simulink model "model_compatible"  (Simulink 7.5)
(part 1 of 2)
settings: Solver=ode45  StartTime=0.0  StopTime=10.0  RelTol=1e-3
libraries: powerlib x223
settings Model: Creator=lej  LastModifiedBy=epezhman  CovModelRefEnable=off
settings DataIOCC: SaveFormat=StructureWithTime
settings OptimizationCC: ExpressionDepthLimit=128
settings DebuggingCC: UnderspecifiedInitializationDetection=Simplified  MergeDetectMultiDrivingBlocksExec=error  SolverPrmCheckMsg=none  FcnCallInpInsideContextMsg=Enable All  StateNameClashWarn=none
settings HardwareCC: ProdIntDivRoundTo=Zero  ProdEndianess=LittleEndian  ProdHWDeviceType=Specified
settings CodeAppCC: CustomSymbolStrType=$N$R$M_T
settings GRTTargetCC: TargetFunctionLibrary=C89/C90 (ANSI)  GeneratePreprocessorConditionals=Use local settings

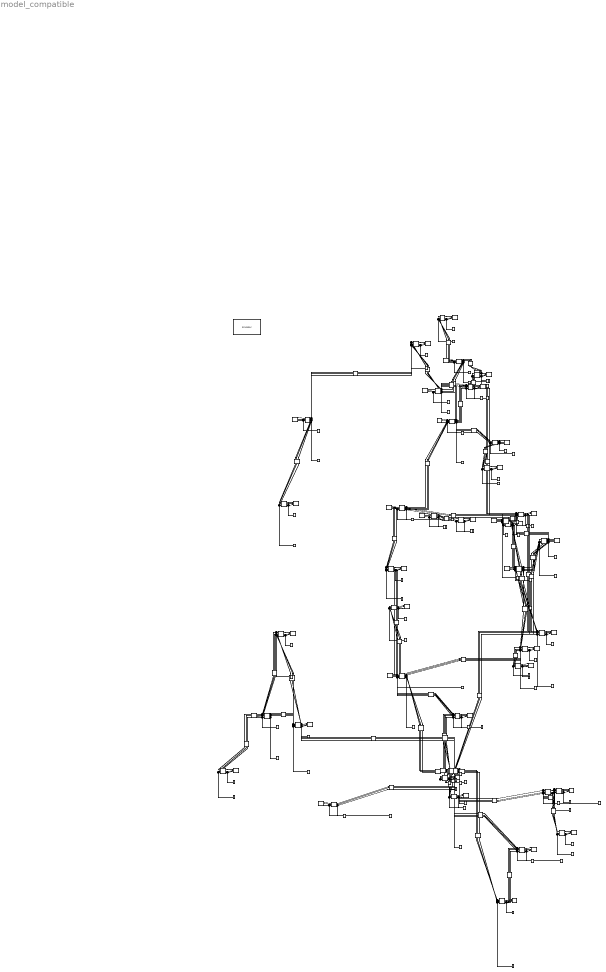
== system model_compatible ==
  note: 150000 Volts Power Line
  note: 225000 Volts Power Line
  DIV_225_Kv_MORNAGUIA_(_MNIHLA_1_BIR_MCHARGA)_CN_129996167_225000_CN_125504235_225000 : powerlib/Elements/Distributed Parameters Line  Phases=3  Frequency=50  Resistance=[0.01273 0.3864]  Inductance="[0.9337e-3  4.1264e-3]"  Capacitance=[12.74e-9 7.751e-9]  Length=112.5736  x1=[8.73114913702011e-11 380000 380000;314.159265358979 314.159265358979 314.159265358979;-0.177670123217348 0.415246442777429 -1.15554988401747]  x2=[1.26090477118469e-09 381852.398472139 381852.398472139;314.159265358979 314.159265358979 314.159265358979;-1.41941675517191 0.415007521738739 -1.15578880505616]  x3=[1.07663708898761e-11 1405.24743813465 1405.24743813466;314.159265358979 314.159265358979 314.159265358979;-2.70558821102223 0.316110507002444 -1.25468581979246]  x4=[8.62234243168895e-12 1405.96374414071 1405.9637441407;314.159265358979 314.159265358979 314.159265358979;0.245769282942371 0.405640215255436 -1.16515611153945]  x5=0.000565541566995742  V1=ones(3,3)  V2=ones(3,3)  I1=ones(3,3)  I2=ones(3,3)  nHarmo=1  Measurements=None
  G_93164455_ : powerlib/Electrical Sources/Three-Phase Source  InternalConnection=Yg  VoltagePhases=off  Voltage=225000  PhaseAngle=0  Voltage_phases=[ 1 1 1]*380000  PhaseAngles_phases=[ 0 0 0]  Frequency=50  NonIdealSource=on  SpecifyImpedance=off  Resistance=0.8929  Inductance=16.58e-3  ShortCircuitLevel=100e6  BaseVoltage=225000  XRratio=7  BusType=swing  Pref=10e3  Qref=0  Prefabc=[3333.33 3333.33 3333.33]  Qrefabc=[0 0 0]  Qmin=-inf  Qmax=inf
  LIGNE_150_KV_METLAOUI_DIV_MDHILLA_CN_206389818_150000_CN_206449367_150000 : powerlib/Elements/Distributed Parameters Line  Phases=3  Frequency=50  Resistance=[0.01273 0.3864]  Inductance="[0.9337e-3  4.1264e-3]"  Capacitance=[12.74e-9 7.751e-9]  Length=32.7201  x1=[8.73114913702011e-11 380000 380000;314.159265358979 314.159265358979 314.159265358979;-0.177670123217348 0.415246442777429 -1.15554988401747]  x2=[1.26090477118469e-09 381852.398472139 381852.398472139;314.159265358979 314.159265358979 314.159265358979;-1.41941675517191 0.415007521738739 -1.15578880505616]  x3=[1.07663708898761e-11 1405.24743813465 1405.24743813466;314.159265358979 314.159265358979 314.159265358979;-2.70558821102223 0.316110507002444 -1.25468581979246]  x4=[8.62234243168895e-12 1405.96374414071 1405.9637441407;314.159265358979 314.159265358979 314.159265358979;0.245769282942371 0.405640215255436 -1.16515611153945]  x5=0.000565541566995742  V1=ones(3,3)  V2=ones(3,3)  I1=ones(3,3)  I2=ones(3,3)  nHarmo=1  Measurements=None
  LIGNE_150_KV_METLAOUI_TOZEUR_CN_207339172_150000_CN_206389818_150000 : powerlib/Elements/Distributed Parameters Line  Phases=3  Frequency=50  Resistance=[0.01273 0.3864]  Inductance="[0.9337e-3  4.1264e-3]"  Capacitance=[12.74e-9 7.751e-9]  Length=61.5655  x1=[8.73114913702011e-11 380000 380000;314.159265358979 314.159265358979 314.159265358979;-0.177670123217348 0.415246442777429 -1.15554988401747]  x2=[1.26090477118469e-09 381852.398472139 381852.398472139;314.159265358979 314.159265358979 314.159265358979;-1.41941675517191 0.415007521738739 -1.15578880505616]  x3=[1.07663708898761e-11 1405.24743813465 1405.24743813466;314.159265358979 314.159265358979 314.159265358979;-2.70558821102223 0.316110507002444 -1.25468581979246]  x4=[8.62234243168895e-12 1405.96374414071 1405.9637441407;314.159265358979 314.159265358979 314.159265358979;0.245769282942371 0.405640215255436 -1.16515611153945]  x5=0.000565541566995742  V1=ones(3,3)  V2=ones(3,3)  I1=ones(3,3)  I2=ones(3,3)  nHarmo=1  Measurements=None
  LIGNE_150_Kv_BOUCHEMMA_CIMENTERIE_DE_GABES_CN_322419513_150000_CN_189193656_150000 : powerlib/Elements/Distributed Parameters Line  Phases=3  Frequency=50  Resistance=[0.01273 0.3864]  Inductance="[0.9337e-3  4.1264e-3]"  Capacitance=[12.74e-9 7.751e-9]  Length=6.701  x1=[8.73114913702011e-11 380000 380000;314.159265358979 314.159265358979 314.159265358979;-0.177670123217348 0.415246442777429 -1.15554988401747]  x2=[1.26090477118469e-09 381852.398472139 381852.398472139;314.159265358979 314.159265358979 314.159265358979;-1.41941675517191 0.415007521738739 -1.15578880505616]  x3=[1.07663708898761e-11 1405.24743813465 1405.24743813466;314.159265358979 314.159265358979 314.159265358979;-2.70558821102223 0.316110507002444 -1.25468581979246]  x4=[8.62234243168895e-12 1405.96374414071 1405.9637441407;314.159265358979 314.159265358979 314.159265358979;0.245769282942371 0.405640215255436 -1.16515611153945]  x5=0.000565541566995742  V1=ones(3,3)  V2=ones(3,3)  I1=ones(3,3)  I2=ones(3,3)  nHarmo=1  Measurements=None
  LIGNE_150_Kv_BOUCHEMMA_GABES_SUD_CN_189193656_150000_CN_242392536_150000 : powerlib/Elements/Distributed Parameters Line  Phases=3  Frequency=50  Resistance=[0.01273 0.3864]  Inductance="[0.9337e-3  4.1264e-3]"  Capacitance=[12.74e-9 7.751e-9]  Length=21.5599  x1=[8.73114913702011e-11 380000 380000;314.159265358979 314.159265358979 314.159265358979;-0.177670123217348 0.415246442777429 -1.15554988401747]  x2=[1.26090477118469e-09 381852.398472139 381852.398472139;314.159265358979 314.159265358979 314.159265358979;-1.41941675517191 0.415007521738739 -1.15578880505616]  x3=[1.07663708898761e-11 1405.24743813465 1405.24743813466;314.159265358979 314.159265358979 314.159265358979;-2.70558821102223 0.316110507002444 -1.25468581979246]  x4=[8.62234243168895e-12 1405.96374414071 1405.9637441407;314.159265358979 314.159265358979 314.159265358979;0.245769282942371 0.405640215255436 -1.16515611153945]  x5=0.000565541566995742  V1=ones(3,3)  V2=ones(3,3)  I1=ones(3,3)  I2=ones(3,3)  nHarmo=1  Measurements=None
  LIGNE_150_Kv_BOUCHEMMA_KEBILI_CN_189193656_150000_CN_253586233_150000 : powerlib/Elements/Distributed Parameters Line  Phases=3  Frequency=50  Resistance=[0.01273 0.3864]  Inductance="[0.9337e-3  4.1264e-3]"  Capacitance=[12.74e-9 7.751e-9]  Length=83.1245  x1=[8.73114913702011e-11 380000 380000;314.159265358979 314.159265358979 314.159265358979;-0.177670123217348 0.415246442777429 -1.15554988401747]  x2=[1.26090477118469e-09 381852.398472139 381852.398472139;314.159265358979 314.159265358979 314.159265358979;-1.41941675517191 0.415007521738739 -1.15578880505616]  x3=[1.07663708898761e-11 1405.24743813465 1405.24743813466;314.159265358979 314.159265358979 314.159265358979;-2.70558821102223 0.316110507002444 -1.25468581979246]  x4=[8.62234243168895e-12 1405.96374414071 1405.9637441407;314.159265358979 314.159265358979 314.159265358979;0.245769282942371 0.405640215255436 -1.16515611153945]  x5=0.000565541566995742  V1=ones(3,3)  V2=ones(3,3)  I1=ones(3,3)  I2=ones(3,3)  nHarmo=1  Measurements=None
  LIGNE_150_Kv_DIV_SKHIRA_CN_202286224_150000_CN_189193656_150000 : powerlib/Elements/Distributed Parameters Line  Phases=3  Frequency=50  Resistance=[0.01273 0.3864]  Inductance="[0.9337e-3  4.1264e-3]"  Capacitance=[12.74e-9 7.751e-9]  Length=63.8559  x1=[8.73114913702011e-11 380000 380000;314.159265358979 314.159265358979 314.159265358979;-0.177670123217348 0.415246442777429 -1.15554988401747]  x2=[1.26090477118469e-09 381852.398472139 381852.398472139;314.159265358979 314.159265358979 314.159265358979;-1.41941675517191 0.415007521738739 -1.15578880505616]  x3=[1.07663708898761e-11 1405.24743813465 1405.24743813466;314.159265358979 314.159265358979 314.159265358979;-2.70558821102223 0.316110507002444 -1.25468581979246]  x4=[8.62234243168895e-12 1405.96374414071 1405.9637441407;314.159265358979 314.159265358979 314.159265358979;0.245769282942371 0.405640215255436 -1.16515611153945]  x5=0.000565541566995742  V1=ones(3,3)  V2=ones(3,3)  I1=ones(3,3)  I2=ones(3,3)  nHarmo=1  Measurements=None
  LIGNE_150_Kv_DIV_SKHIRA_CN_202286224_150000_CN_201812735_150000 : powerlib/Elements/Distributed Parameters Line  Phases=3  Frequency=50  Resistance=[0.01273 0.3864]  Inductance="[0.9337e-3  4.1264e-3]"  Capacitance=[12.74e-9 7.751e-9]  Length=60.8483  x1=[8.73114913702011e-11 380000 380000;314.159265358979 314.159265358979 314.159265358979;-0.177670123217348 0.415246442777429 -1.15554988401747]  x2=[1.26090477118469e-09 381852.398472139 381852.398472139;314.159265358979 314.159265358979 314.159265358979;-1.41941675517191 0.415007521738739 -1.15578880505616]  x3=[1.07663708898761e-11 1405.24743813465 1405.24743813466;314.159265358979 314.159265358979 314.159265358979;-2.70558821102223 0.316110507002444 -1.25468581979246]  x4=[8.62234243168895e-12 1405.96374414071 1405.9637441407;314.159265358979 314.159265358979 314.159265358979;0.245769282942371 0.405640215255436 -1.16515611153945]  x5=0.000565541566995742  V1=ones(3,3)  V2=ones(3,3)  I1=ones(3,3)  I2=ones(3,3)  nHarmo=1  Measurements=None
  LIGNE_150_Kv_DIV_SKHIRA_CN_202286224_150000_CN_242390602_150000 : powerlib/Elements/Distributed Parameters Line  Phases=3  Frequency=50  Resistance=[0.01273 0.3864]  Inductance="[0.9337e-3  4.1264e-3]"  Capacitance=[12.74e-9 7.751e-9]  Length=66.6914  x1=[8.73114913702011e-11 380000 380000;314.159265358979 314.159265358979 314.159265358979;-0.177670123217348 0.415246442777429 -1.15554988401747]  x2=[1.26090477118469e-09 381852.398472139 381852.398472139;314.159265358979 314.159265358979 314.159265358979;-1.41941675517191 0.415007521738739 -1.15578880505616]  x3=[1.07663708898761e-11 1405.24743813465 1405.24743813466;314.159265358979 314.159265358979 314.159265358979;-2.70558821102223 0.316110507002444 -1.25468581979246]  x4=[8.62234243168895e-12 1405.96374414071 1405.9637441407;314.159265358979 314.159265358979 314.159265358979;0.245769282942371 0.405640215255436 -1.16515611153945]  x5=0.000565541566995742  V1=ones(3,3)  V2=ones(3,3)  I1=ones(3,3)  I2=ones(3,3)  nHarmo=1  Measurements=None
  LIGNE_150_Kv_ENFIDHA_DIV_BOUFICHA_CN_131220525_150000_CN_106469430_150000 : powerlib/Elements/Distributed Parameters Line  Phases=3  Frequency=50  Resistance=[0.01273 0.3864]  Inductance="[0.9337e-3  4.1264e-3]"  Capacitance=[12.74e-9 7.751e-9]  Length=29.2926  x1=[8.73114913702011e-11 380000 380000;314.159265358979 314.159265358979 314.159265358979;-0.177670123217348 0.415246442777429 -1.15554988401747]  x2=[1.26090477118469e-09 381852.398472139 381852.398472139;314.159265358979 314.159265358979 314.159265358979;-1.41941675517191 0.415007521738739 -1.15578880505616]  x3=[1.07663708898761e-11 1405.24743813465 1405.24743813466;314.159265358979 314.159265358979 314.159265358979;-2.70558821102223 0.316110507002444 -1.25468581979246]  x4=[8.62234243168895e-12 1405.96374414071 1405.9637441407;314.159265358979 314.159265358979 314.159265358979;0.245769282942371 0.405640215255436 -1.16515611153945]  x5=0.000565541566995742  V1=ones(3,3)  V2=ones(3,3)  I1=ones(3,3)  I2=ones(3,3)  nHarmo=1  Measurements=None
  LIGNE_150_Kv_MEKNASSY_HAJEB_LAYOUN_CN_224417135_225000_CN_201812735_225000 : powerlib/Elements/Distributed Parameters Line  Phases=3  Frequency=50  Resistance=[0.01273 0.3864]  Inductance="[0.9337e-3  4.1264e-3]"  Capacitance=[12.74e-9 7.751e-9]  Length=81.6177  x1=[8.73114913702011e-11 380000 380000;314.159265358979 314.159265358979 314.159265358979;-0.177670123217348 0.415246442777429 -1.15554988401747]  x2=[1.26090477118469e-09 381852.398472139 381852.398472139;314.159265358979 314.159265358979 314.159265358979;-1.41941675517191 0.415007521738739 -1.15578880505616]  x3=[1.07663708898761e-11 1405.24743813465 1405.24743813466;314.159265358979 314.159265358979 314.159265358979;-2.70558821102223 0.316110507002444 -1.25468581979246]  x4=[8.62234243168895e-12 1405.96374414071 1405.9637441407;314.159265358979 314.159265358979 314.159265358979;0.245769282942371 0.405640215255436 -1.16515611153945]  x5=0.000565541566995742  V1=ones(3,3)  V2=ones(3,3)  I1=ones(3,3)  I2=ones(3,3)  nHarmo=1  Measurements=None
  LIGNE_150_Kv_MEKNASSY_SIDI_BOUZID_CN_174150822_150000_CN_201812735_150000 : powerlib/Elements/Distributed Parameters Line  Phases=3  Frequency=50  Resistance=[0.01273 0.3864]  Inductance="[0.9337e-3  4.1264e-3]"  Capacitance=[12.74e-9 7.751e-9]  Length=56.6763  x1=[8.73114913702011e-11 380000 380000;314.159265358979 314.159265358979 314.159265358979;-0.177670123217348 0.415246442777429 -1.15554988401747]  x2=[1.26090477118469e-09 381852.398472139 381852.398472139;314.159265358979 314.159265358979 314.159265358979;-1.41941675517191 0.415007521738739 -1.15578880505616]  x3=[1.07663708898761e-11 1405.24743813465 1405.24743813466;314.159265358979 314.159265358979 314.159265358979;-2.70558821102223 0.316110507002444 -1.25468581979246]  x4=[8.62234243168895e-12 1405.96374414071 1405.9637441407;314.159265358979 314.159265358979 314.159265358979;0.245769282942371 0.405640215255436 -1.16515611153945]  x5=0.000565541566995742  V1=ones(3,3)  V2=ones(3,3)  I1=ones(3,3)  I2=ones(3,3)  nHarmo=1  Measurements=None
  LIGNE_150_Kv_MOKNINE_ELJEM_CN_178549814_150000_CN_178326515_150000 : powerlib/Elements/Distributed Parameters Line  Phases=3  Frequency=50  Resistance=[0.01273 0.3864]  Inductance="[0.9337e-3  4.1264e-3]"  Capacitance=[12.74e-9 7.751e-9]  Length=33.8315  x1=[8.73114913702011e-11 380000 380000;314.159265358979 314.159265358979 314.159265358979;-0.177670123217348 0.415246442777429 -1.15554988401747]  x2=[1.26090477118469e-09 381852.398472139 381852.398472139;314.159265358979 314.159265358979 314.159265358979;-1.41941675517191 0.415007521738739 -1.15578880505616]  x3=[1.07663708898761e-11 1405.24743813465 1405.24743813466;314.159265358979 314.159265358979 314.159265358979;-2.70558821102223 0.316110507002444 -1.25468581979246]  x4=[8.62234243168895e-12 1405.96374414071 1405.9637441407;314.159265358979 314.159265358979 314.159265358979;0.245769282942371 0.405640215255436 -1.16515611153945]  x5=0.000565541566995742  V1=ones(3,3)  V2=ones(3,3)  I1=ones(3,3)  I2=ones(3,3)  nHarmo=1  Measurements=None
  LIGNE_150_Kv_MSAKEN_NORD_MSAKEN_3_CN_28943745_150000_CN_130775787_150000 : powerlib/Elements/Distributed Parameters Line  Phases=3  Frequency=50  Resistance=[0.01273 0.3864]  Inductance="[0.9337e-3  4.1264e-3]"  Capacitance=[12.74e-9 7.751e-9]  Length=2.304  x1=[8.73114913702011e-11 380000 380000;314.159265358979 314.159265358979 314.159265358979;-0.177670123217348 0.415246442777429 -1.15554988401747]  x2=[1.26090477118469e-09 381852.398472139 381852.398472139;314.159265358979 314.159265358979 314.159265358979;-1.41941675517191 0.415007521738739 -1.15578880505616]  x3=[1.07663708898761e-11 1405.24743813465 1405.24743813466;314.159265358979 314.159265358979 314.159265358979;-2.70558821102223 0.316110507002444 -1.25468581979246]  x4=[8.62234243168895e-12 1405.96374414071 1405.9637441407;314.159265358979 314.159265358979 314.159265358979;0.245769282942371 0.405640215255436 -1.16515611153945]  x5=0.000565541566995742  V1=ones(3,3)  V2=ones(3,3)  I1=ones(3,3)  I2=ones(3,3)  nHarmo=1  Measurements=None
  LIGNE_150_Kv_SFAX_SIDI_MANSOUR_CN_178543491_150000_CN_178549814_150000 : powerlib/Elements/Distributed Parameters Line  Phases=3  Frequency=50  Resistance=[0.01273 0.3864]  Inductance="[0.9337e-3  4.1264e-3]"  Capacitance=[12.74e-9 7.751e-9]  Length=65.4863  x1=[8.73114913702011e-11 380000 380000;314.159265358979 314.159265358979 314.159265358979;-0.177670123217348 0.415246442777429 -1.15554988401747]  x2=[1.26090477118469e-09 381852.398472139 381852.398472139;314.159265358979 314.159265358979 314.159265358979;-1.41941675517191 0.415007521738739 -1.15578880505616]  x3=[1.07663708898761e-11 1405.24743813465 1405.24743813466;314.159265358979 314.159265358979 314.159265358979;-2.70558821102223 0.316110507002444 -1.25468581979246]  x4=[8.62234243168895e-12 1405.96374414071 1405.9637441407;314.159265358979 314.159265358979 314.159265358979;0.245769282942371 0.405640215255436 -1.16515611153945]  x5=0.000565541566995742  V1=ones(3,3)  V2=ones(3,3)  I1=ones(3,3)  I2=ones(3,3)  nHarmo=1  Measurements=None
  LIGNE_150_Kv_SFAX_THYNA_CN_178543491_150000_CN_178547287_150000 : powerlib/Elements/Distributed Parameters Line  Phases=3  Frequency=50  Resistance=[0.01273 0.3864]  Inductance="[0.9337e-3  4.1264e-3]"  Capacitance=[12.74e-9 7.751e-9]  Length=23.3899  x1=[8.73114913702011e-11 380000 380000;314.159265358979 314.159265358979 314.159265358979;-0.177670123217348 0.415246442777429 -1.15554988401747]  x2=[1.26090477118469e-09 381852.398472139 381852.398472139;314.159265358979 314.159265358979 314.159265358979;-1.41941675517191 0.415007521738739 -1.15578880505616]  x3=[1.07663708898761e-11 1405.24743813465 1405.24743813466;314.159265358979 314.159265358979 314.159265358979;-2.70558821102223 0.316110507002444 -1.25468581979246]  x4=[8.62234243168895e-12 1405.96374414071 1405.9637441407;314.159265358979 314.159265358979 314.159265358979;0.245769282942371 0.405640215255436 -1.16515611153945]  x5=0.000565541566995742  V1=ones(3,3)  V2=ones(3,3)  I1=ones(3,3)  I2=ones(3,3)  nHarmo=1  Measurements=None
  LIGNE_150_Kv_SFAX_THYNA_CN_178543491_150000_CN_201812735_150000 : powerlib/Elements/Distributed Parameters Line  Phases=3  Frequency=50  Resistance=[0.01273 0.3864]  Inductance="[0.9337e-3  4.1264e-3]"  Capacitance=[12.74e-9 7.751e-9]  Length=21.1003  x1=[8.73114913702011e-11 380000 380000;314.159265358979 314.159265358979 314.159265358979;-0.177670123217348 0.415246442777429 -1.15554988401747]  x2=[1.26090477118469e-09 381852.398472139 381852.398472139;314.159265358979 314.159265358979 314.159265358979;-1.41941675517191 0.415007521738739 -1.15578880505616]  x3=[1.07663708898761e-11 1405.24743813465 1405.24743813466;314.159265358979 314.159265358979 314.159265358979;-2.70558821102223 0.316110507002444 -1.25468581979246]  x4=[8.62234243168895e-12 1405.96374414071 1405.9637441407;314.159265358979 314.159265358979 314.159265358979;0.245769282942371 0.405640215255436 -1.16515611153945]  x5=0.000565541566995742  V1=ones(3,3)  V2=ones(3,3)  I1=ones(3,3)  I2=ones(3,3)  nHarmo=1  Measurements=None
  LIGNE_150_Kv_SOUSSE_MSAKEN_NORD_CN_28943745_150000_CN_111375430_150000 : powerlib/Elements/Distributed Parameters Line  Phases=3  Frequency=50  Resistance=[0.01273 0.3864]  Inductance="[0.9337e-3  4.1264e-3]"  Capacitance=[12.74e-9 7.751e-9]  Length=13.399  x1=[8.73114913702011e-11 380000 380000;314.159265358979 314.159265358979 314.159265358979;-0.177670123217348 0.415246442777429 -1.15554988401747]  x2=[1.26090477118469e-09 381852.398472139 381852.398472139;314.159265358979 314.159265358979 314.159265358979;-1.41941675517191 0.415007521738739 -1.15578880505616]  x3=[1.07663708898761e-11 1405.24743813465 1405.24743813466;314.159265358979 314.159265358979 314.159265358979;-2.70558821102223 0.316110507002444 -1.25468581979246]  x4=[8.62234243168895e-12 1405.96374414071 1405.9637441407;314.159265358979 314.159265358979 314.159265358979;0.245769282942371 0.405640215255436 -1.16515611153945]  x5=0.000565541566995742  V1=ones(3,3)  V2=ones(3,3)  I1=ones(3,3)  I2=ones(3,3)  nHarmo=1  Measurements=None
  LIGNE_150_Kv__MSAKEN_ELJEM_CN_178549814_150000_CN_130775787_150000 : powerlib/Elements/Distributed Parameters Line  Phases=3  Frequency=50  Resistance=[0.01273 0.3864]  Inductance="[0.9337e-3  4.1264e-3]"  Capacitance=[12.74e-9 7.751e-9]  Length=37.6275  x1=[8.73114913702011e-11 380000 380000;314.159265358979 314.159265358979 314.159265358979;-0.177670123217348 0.415246442777429 -1.15554988401747]  x2=[1.26090477118469e-09 381852.398472139 381852.398472139;314.159265358979 314.159265358979 314.159265358979;-1.41941675517191 0.415007521738739 -1.15578880505616]  x3=[1.07663708898761e-11 1405.24743813465 1405.24743813466;314.159265358979 314.159265358979 314.159265358979;-2.70558821102223 0.316110507002444 -1.25468581979246]  x4=[8.62234243168895e-12 1405.96374414071 1405.9637441407;314.159265358979 314.159265358979 314.159265358979;0.245769282942371 0.405640215255436 -1.16515611153945]  x5=0.000565541566995742  V1=ones(3,3)  V2=ones(3,3)  I1=ones(3,3)  I2=ones(3,3)  nHarmo=1  Measurements=None
  LIGNE_225_Kv_BOUCHEMMA_MEKNASSY_CN_189193646_225000_CN_201812735_225000 : powerlib/Elements/Distributed Parameters Line  Phases=3  Frequency=50  Resistance=[0.01273 0.3864]  Inductance="[0.9337e-3  4.1264e-3]"  Capacitance=[12.74e-9 7.751e-9]  Length=7.3111  x1=[8.73114913702011e-11 380000 380000;314.159265358979 314.159265358979 314.159265358979;-0.177670123217348 0.415246442777429 -1.15554988401747]  x2=[1.26090477118469e-09 381852.398472139 381852.398472139;314.159265358979 314.159265358979 314.159265358979;-1.41941675517191 0.415007521738739 -1.15578880505616]  x3=[1.07663708898761e-11 1405.24743813465 1405.24743813466;314.159265358979 314.159265358979 314.159265358979;-2.70558821102223 0.316110507002444 -1.25468581979246]  x4=[8.62234243168895e-12 1405.96374414071 1405.9637441407;314.159265358979 314.159265358979 314.159265358979;0.245769282942371 0.405640215255436 -1.16515611153945]  x5=0.000565541566995742  V1=ones(3,3)  V2=ones(3,3)  I1=ones(3,3)  I2=ones(3,3)  nHarmo=1  Measurements=None
  LIGNE_225_Kv_BOUCHEMMA_TATAOUINE_CN_189193646_225000_CN_180615776_225000 : powerlib/Elements/Distributed Parameters Line  Phases=3  Frequency=50  Resistance=[0.01273 0.3864]  Inductance="[0.9337e-3  4.1264e-3]"  Capacitance=[12.74e-9 7.751e-9]  Length=34.803  x1=[8.73114913702011e-11 380000 380000;314.159265358979 314.159265358979 314.159265358979;-0.177670123217348 0.415246442777429 -1.15554988401747]  x2=[1.26090477118469e-09 381852.398472139 381852.398472139;314.159265358979 314.159265358979 314.159265358979;-1.41941675517191 0.415007521738739 -1.15578880505616]  x3=[1.07663708898761e-11 1405.24743813465 1405.24743813466;314.159265358979 314.159265358979 314.159265358979;-2.70558821102223 0.316110507002444 -1.25468581979246]  x4=[8.62234243168895e-12 1405.96374414071 1405.9637441407;314.159265358979 314.159265358979 314.159265358979;0.245769282942371 0.405640215255436 -1.16515611153945]  x5=0.000565541566995742  V1=ones(3,3)  V2=ones(3,3)  I1=ones(3,3)  I2=ones(3,3)  nHarmo=1  Measurements=None
  LIGNE_225_Kv_KAIROUAN_CIMENTERIE_CN_242398869_225000_CN_226848748_225000 : powerlib/Elements/Distributed Parameters Line  Phases=3  Frequency=50  Resistance=[0.01273 0.3864]  Inductance="[0.9337e-3  4.1264e-3]"  Capacitance=[12.74e-9 7.751e-9]  Length=23.7865  x1=[8.73114913702011e-11 380000 380000;314.159265358979 314.159265358979 314.159265358979;-0.177670123217348 0.415246442777429 -1.15554988401747]  x2=[1.26090477118469e-09 381852.398472139 381852.398472139;314.159265358979 314.159265358979 314.159265358979;-1.41941675517191 0.415007521738739 -1.15578880505616]  x3=[1.07663708898761e-11 1405.24743813465 1405.24743813466;314.159265358979 314.159265358979 314.159265358979;-2.70558821102223 0.316110507002444 -1.25468581979246]  x4=[8.62234243168895e-12 1405.96374414071 1405.9637441407;314.159265358979 314.159265358979 314.159265358979;0.245769282942371 0.405640215255436 -1.16515611153945]  x5=0.000565541566995742  V1=ones(3,3)  V2=ones(3,3)  I1=ones(3,3)  I2=ones(3,3)  nHarmo=1  Measurements=None
  LIGNE_225_Kv_MEDENINE_TATAOUINE_CN_180615776_225000_CN_180611326_225000 : powerlib/Elements/Distributed Parameters Line  Phases=3  Frequency=50  Resistance=[0.01273 0.3864]  Inductance="[0.9337e-3  4.1264e-3]"  Capacitance=[12.74e-9 7.751e-9]  Length=45.5395  x1=[8.73114913702011e-11 380000 380000;314.159265358979 314.159265358979 314.159265358979;-0.177670123217348 0.415246442777429 -1.15554988401747]  x2=[1.26090477118469e-09 381852.398472139 381852.398472139;314.159265358979 314.159265358979 314.159265358979;-1.41941675517191 0.415007521738739 -1.15578880505616]  x3=[1.07663708898761e-11 1405.24743813465 1405.24743813466;314.159265358979 314.159265358979 314.159265358979;-2.70558821102223 0.316110507002444 -1.25468581979246]  x4=[8.62234243168895e-12 1405.96374414071 1405.9637441407;314.159265358979 314.159265358979 314.159265358979;0.245769282942371 0.405640215255436 -1.16515611153945]  x5=0.000565541566995742  V1=ones(3,3)  V2=ones(3,3)  I1=ones(3,3)  I2=ones(3,3)  nHarmo=1  Measurements=None
  LIGNE_225_Kv_MNIHLA_1_MENZEL_JEMIL_CN_101404944_225000_CN_178494278_225000 : powerlib/Elements/Distributed Parameters Line  Phases=3  Frequency=50  Resistance=[0.01273 0.3864]  Inductance="[0.9337e-3  4.1264e-3]"  Capacitance=[12.74e-9 7.751e-9]  Length=40.4216  x1=[8.73114913702011e-11 380000 380000;314.159265358979 314.159265358979 314.159265358979;-0.177670123217348 0.415246442777429 -1.15554988401747]  x2=[1.26090477118469e-09 381852.398472139 381852.398472139;314.159265358979 314.159265358979 314.159265358979;-1.41941675517191 0.415007521738739 -1.15578880505616]  x3=[1.07663708898761e-11 1405.24743813465 1405.24743813466;314.159265358979 314.159265358979 314.159265358979;-2.70558821102223 0.316110507002444 -1.25468581979246]  x4=[8.62234243168895e-12 1405.96374414071 1405.9637441407;314.159265358979 314.159265358979 314.159265358979;0.245769282942371 0.405640215255436 -1.16515611153945]  x5=0.000565541566995742  V1=ones(3,3)  V2=ones(3,3)  I1=ones(3,3)  I2=ones(3,3)  nHarmo=1  Measurements=None
  LIGNE_225_Kv_NAASAN_BIR_MCHARGA_CN_173531194_225000_CN_125504235_225000 : powerlib/Elements/Distributed Parameters Line  Phases=3  Frequency=50  Resistance=[0.01273 0.3864]  Inductance="[0.9337e-3  4.1264e-3]"  Capacitance=[12.74e-9 7.751e-9]  Length=32.5012  x1=[8.73114913702011e-11 380000 380000;314.159265358979 314.159265358979 314.159265358979;-0.177670123217348 0.415246442777429 -1.15554988401747]  x2=[1.26090477118469e-09 381852.398472139 381852.398472139;314.159265358979 314.159265358979 314.159265358979;-1.41941675517191 0.415007521738739 -1.15578880505616]  x3=[1.07663708898761e-11 1405.24743813465 1405.24743813466;314.159265358979 314.159265358979 314.159265358979;-2.70558821102223 0.316110507002444 -1.25468581979246]  x4=[8.62234243168895e-12 1405.96374414071 1405.9637441407;314.159265358979 314.159265358979 314.159265358979;0.245769282942371 0.405640215255436 -1.16515611153945]  x5=0.000565541566995742  V1=ones(3,3)  V2=ones(3,3)  I1=ones(3,3)  I2=ones(3,3)  nHarmo=1  Measurements=None
  LIGNE_225_Kv_OUESLATIA_BIR_MCHARGA_CN_224416644_225000_CN_173531194_225000 : powerlib/Elements/Distributed Parameters Line  Phases=3  Frequency=50  Resistance=[0.01273 0.3864]  Inductance="[0.9337e-3  4.1264e-3]"  Capacitance=[12.74e-9 7.751e-9]  Length=80.5638  x1=[8.73114913702011e-11 380000 380000;314.159265358979 314.159265358979 314.159265358979;-0.177670123217348 0.415246442777429 -1.15554988401747]  x2=[1.26090477118469e-09 381852.398472139 381852.398472139;314.159265358979 314.159265358979 314.159265358979;-1.41941675517191 0.415007521738739 -1.15578880505616]  x3=[1.07663708898761e-11 1405.24743813465 1405.24743813466;314.159265358979 314.159265358979 314.159265358979;-2.70558821102223 0.316110507002444 -1.25468581979246]  x4=[8.62234243168895e-12 1405.96374414071 1405.9637441407;314.159265358979 314.159265358979 314.159265358979;0.245769282942371 0.405640215255436 -1.16515611153945]  x5=0.000565541566995742  V1=ones(3,3)  V2=ones(3,3)  I1=ones(3,3)  I2=ones(3,3)  nHarmo=1  Measurements=None
  LIGNE_225_Kv_OUESLATIA_HAJEB_LAYOUN_CN_224416644_225000_CN_224417135_225000 : powerlib/Elements/Distributed Parameters Line  Phases=3  Frequency=50  Resistance=[0.01273 0.3864]  Inductance="[0.9337e-3  4.1264e-3]"  Capacitance=[12.74e-9 7.751e-9]  Length=50.1058  x1=[8.73114913702011e-11 380000 380000;314.159265358979 314.159265358979 314.159265358979;-0.177670123217348 0.415246442777429 -1.15554988401747]  x2=[1.26090477118469e-09 381852.398472139 381852.398472139;314.159265358979 314.159265358979 314.159265358979;-1.41941675517191 0.415007521738739 -1.15578880505616]  x3=[1.07663708898761e-11 1405.24743813465 1405.24743813466;314.159265358979 314.159265358979 314.159265358979;-2.70558821102223 0.316110507002444 -1.25468581979246]  x4=[8.62234243168895e-12 1405.96374414071 1405.9637441407;314.159265358979 314.159265358979 314.159265358979;0.245769282942371 0.405640215255436 -1.16515611153945]  x5=0.000565541566995742  V1=ones(3,3)  V2=ones(3,3)  I1=ones(3,3)  I2=ones(3,3)  nHarmo=1  Measurements=None
  LIGNE_225_Kv_RADES_NAASAN_CN_93263381_225000_CN_125504235_225000 : powerlib/Elements/Distributed Parameters Line  Phases=3  Frequency=50  Resistance=[0.01273 0.3864]  Inductance="[0.9337e-3  4.1264e-3]"  Capacitance=[12.74e-9 7.751e-9]  Length=15.3726  x1=[8.73114913702011e-11 380000 380000;314.159265358979 314.159265358979 314.159265358979;-0.177670123217348 0.415246442777429 -1.15554988401747]  x2=[1.26090477118469e-09 381852.398472139 381852.398472139;314.159265358979 314.159265358979 314.159265358979;-1.41941675517191 0.415007521738739 -1.15578880505616]  x3=[1.07663708898761e-11 1405.24743813465 1405.24743813466;314.159265358979 314.159265358979 314.159265358979;-2.70558821102223 0.316110507002444 -1.25468581979246]  x4=[8.62234243168895e-12 1405.96374414071 1405.9637441407;314.159265358979 314.159265358979 314.159265358979;0.245769282942371 0.405640215255436 -1.16515611153945]  x5=0.000565541566995742  V1=ones(3,3)  V2=ones(3,3)  I1=ones(3,3)  I2=ones(3,3)  nHarmo=1  Measurements=None
  LIGNE_225_Kv_SIDI_MANSOUR_DIV_MOKNINE_CN_178328237_225000_CN_111375420_225000 : powerlib/Elements/Distributed Parameters Line  Phases=3  Frequency=50  Resistance=[0.01273 0.3864]  Inductance="[0.9337e-3  4.1264e-3]"  Capacitance=[12.74e-9 7.751e-9]  Length=101.3181  x1=[8.73114913702011e-11 380000 380000;314.159265358979 314.159265358979 314.159265358979;-0.177670123217348 0.415246442777429 -1.15554988401747]  x2=[1.26090477118469e-09 381852.398472139 381852.398472139;314.159265358979 314.159265358979 314.159265358979;-1.41941675517191 0.415007521738739 -1.15578880505616]  x3=[1.07663708898761e-11 1405.24743813465 1405.24743813466;314.159265358979 314.159265358979 314.159265358979;-2.70558821102223 0.316110507002444 -1.25468581979246]  x4=[8.62234243168895e-12 1405.96374414071 1405.9637441407;314.159265358979 314.159265358979 314.159265358979;0.245769282942371 0.405640215255436 -1.16515611153945]  x5=0.000565541566995742  V1=ones(3,3)  V2=ones(3,3)  I1=ones(3,3)  I2=ones(3,3)  nHarmo=1  Measurements=None
  LIGNE_225_Kv_SIDI_MANSOUR_DIV_MOKNINE_CN_178328237_225000_CN_178326515_225000 : powerlib/Elements/Distributed Parameters Line  Phases=3  Frequency=50  Resistance=[0.01273 0.3864]  Inductance="[0.9337e-3  4.1264e-3]"  Capacitance=[12.74e-9 7.751e-9]  Length=101.2274  x1=[8.73114913702011e-11 380000 380000;314.159265358979 314.159265358979 314.159265358979;-0.177670123217348 0.415246442777429 -1.15554988401747]  x2=[1.26090477118469e-09 381852.398472139 381852.398472139;314.159265358979 314.159265358979 314.159265358979;-1.41941675517191 0.415007521738739 -1.15578880505616]  x3=[1.07663708898761e-11 1405.24743813465 1405.24743813466;314.159265358979 314.159265358979 314.159265358979;-2.70558821102223 0.316110507002444 -1.25468581979246]  x4=[8.62234243168895e-12 1405.96374414071 1405.9637441407;314.159265358979 314.159265358979 314.159265358979;0.245769282942371 0.405640215255436 -1.16515611153945]  x5=0.000565541566995742  V1=ones(3,3)  V2=ones(3,3)  I1=ones(3,3)  I2=ones(3,3)  nHarmo=1  Measurements=None
  LIGNE_225_Kv_SIDI_MANSOUR_MSAKEN_NORD_CN_28943745_225000_CN_178328237_225000 : powerlib/Elements/Distributed Parameters Line  Phases=3  Frequency=50  Resistance=[0.01273 0.3864]  Inductance="[0.9337e-3  4.1264e-3]"  Capacitance=[12.74e-9 7.751e-9]  Length=81.2863  x1=[8.73114913702011e-11 380000 380000;314.159265358979 314.159265358979 314.159265358979;-0.177670123217348 0.415246442777429 -1.15554988401747]  x2=[1.26090477118469e-09 381852.398472139 381852.398472139;314.159265358979 314.159265358979 314.159265358979;-1.41941675517191 0.415007521738739 -1.15578880505616]  x3=[1.07663708898761e-11 1405.24743813465 1405.24743813466;314.159265358979 314.159265358979 314.159265358979;-2.70558821102223 0.316110507002444 -1.25468581979246]  x4=[8.62234243168895e-12 1405.96374414071 1405.9637441407;314.159265358979 314.159265358979 314.159265358979;0.245769282942371 0.405640215255436 -1.16515611153945]  x5=0.000565541566995742  V1=ones(3,3)  V2=ones(3,3)  I1=ones(3,3)  I2=ones(3,3)  nHarmo=1  Measurements=None
  LIGNE_225_Kv_SOUSSE_NAASAN_CN_111375420_225000_CN_125504235_225000 : powerlib/Elements/Distributed Parameters Line  Phases=3  Frequency=50  Resistance=[0.01273 0.3864]  Inductance="[0.9337e-3  4.1264e-3]"  Capacitance=[12.74e-9 7.751e-9]  Length=80.2922  x1=[8.73114913702011e-11 380000 380000;314.159265358979 314.159265358979 314.159265358979;-0.177670123217348 0.415246442777429 -1.15554988401747]  x2=[1.26090477118469e-09 381852.398472139 381852.398472139;314.159265358979 314.159265358979 314.159265358979;-1.41941675517191 0.415007521738739 -1.15578880505616]  x3=[1.07663708898761e-11 1405.24743813465 1405.24743813466;314.159265358979 314.159265358979 314.159265358979;-2.70558821102223 0.316110507002444 -1.25468581979246]  x4=[8.62234243168895e-12 1405.96374414071 1405.9637441407;314.159265358979 314.159265358979 314.159265358979;0.245769282942371 0.405640215255436 -1.16515611153945]  x5=0.000565541566995742  V1=ones(3,3)  V2=ones(3,3)  I1=ones(3,3)  I2=ones(3,3)  nHarmo=1  Measurements=None
  LIGNE_225_Kv_SOUSSE__MOKNINE_CN_111375430_150000_CN_178326515_150000 : powerlib/Elements/Distributed Parameters Line  Phases=3  Frequency=50  Resistance=[0.01273 0.3864]  Inductance="[0.9337e-3  4.1264e-3]"  Capacitance=[12.74e-9 7.751e-9]  Length=36.4839  x1=[8.73114913702011e-11 380000 380000;314.159265358979 314.159265358979 314.159265358979;-0.177670123217348 0.415246442777429 -1.15554988401747]  x2=[1.26090477118469e-09 381852.398472139 381852.398472139;314.159265358979 314.159265358979 314.159265358979;-1.41941675517191 0.415007521738739 -1.15578880505616]  x3=[1.07663708898761e-11 1405.24743813465 1405.24743813466;314.159265358979 314.159265358979 314.159265358979;-2.70558821102223 0.316110507002444 -1.25468581979246]  x4=[8.62234243168895e-12 1405.96374414071 1405.9637441407;314.159265358979 314.159265358979 314.159265358979;0.245769282942371 0.405640215255436 -1.16515611153945]  x5=0.000565541566995742  V1=ones(3,3)  V2=ones(3,3)  I1=ones(3,3)  I2=ones(3,3)  nHarmo=1  Measurements=None
  LIGNE_225_Kv_TAJEROUIN_JANDOUBA_CN_179549833_225000_CN_173534564_225000 : powerlib/Elements/Distributed Parameters Line  Phases=3  Frequency=50  Resistance=[0.01273 0.3864]  Inductance="[0.9337e-3  4.1264e-3]"  Capacitance=[12.74e-9 7.751e-9]  Length=74.2067  x1=[8.73114913702011e-11 380000 380000;314.159265358979 314.159265358979 314.159265358979;-0.177670123217348 0.415246442777429 -1.15554988401747]  x2=[1.26090477118469e-09 381852.398472139 381852.398472139;314.159265358979 314.159265358979 314.159265358979;-1.41941675517191 0.415007521738739 -1.15578880505616]  x3=[1.07663708898761e-11 1405.24743813465 1405.24743813466;314.159265358979 314.159265358979 314.159265358979;-2.70558821102223 0.316110507002444 -1.25468581979246]  x4=[8.62234243168895e-12 1405.96374414071 1405.9637441407;314.159265358979 314.159265358979 314.159265358979;0.245769282942371 0.405640215255436 -1.16515611153945]  x5=0.000565541566995742  V1=ones(3,3)  V2=ones(3,3)  I1=ones(3,3)  I2=ones(3,3)  nHarmo=1  Measurements=None
  LIGNE_225_Kv__BOUFICHA_ZAGHOUAN_CN_106469430_225000_CN_173531194_225000 : powerlib/Elements/Distributed Parameters Line  Phases=3  Frequency=50  Resistance=[0.01273 0.3864]  Inductance="[0.9337e-3  4.1264e-3]"  Capacitance=[12.74e-9 7.751e-9]  Length=41.8979  x1=[8.73114913702011e-11 380000 380000;314.159265358979 314.159265358979 314.159265358979;-0.177670123217348 0.415246442777429 -1.15554988401747]  x2=[1.26090477118469e-09 381852.398472139 381852.398472139;314.159265358979 314.159265358979 314.159265358979;-1.41941675517191 0.415007521738739 -1.15578880505616]  x3=[1.07663708898761e-11 1405.24743813465 1405.24743813466;314.159265358979 314.159265358979 314.159265358979;-2.70558821102223 0.316110507002444 -1.25468581979246]  x4=[8.62234243168895e-12 1405.96374414071 1405.9637441407;314.159265358979 314.159265358979 314.159265358979;0.245769282942371 0.405640215255436 -1.16515611153945]  x5=0.000565541566995742  V1=ones(3,3)  V2=ones(3,3)  I1=ones(3,3)  I2=ones(3,3)  nHarmo=1  Measurements=None
  LIGNE_400_Kv_JANDOUBA_MATEUR_CN_129996179_225000_CN_173534564_225000 : powerlib/Elements/Distributed Parameters Line  Phases=3  Frequency=50  Resistance=[0.01273 0.3864]  Inductance="[0.9337e-3  4.1264e-3]"  Capacitance=[12.74e-9 7.751e-9]  Length=37.0111  x1=[8.73114913702011e-11 380000 380000;314.159265358979 314.159265358979 314.159265358979;-0.177670123217348 0.415246442777429 -1.15554988401747]  x2=[1.26090477118469e-09 381852.398472139 381852.398472139;314.159265358979 314.159265358979 314.159265358979;-1.41941675517191 0.415007521738739 -1.15578880505616]  x3=[1.07663708898761e-11 1405.24743813465 1405.24743813466;314.159265358979 314.159265358979 314.159265358979;-2.70558821102223 0.316110507002444 -1.25468581979246]  x4=[8.62234243168895e-12 1405.96374414071 1405.9637441407;314.159265358979 314.159265358979 314.159265358979;0.245769282942371 0.405640215255436 -1.16515611153945]  x5=0.000565541566995742  V1=ones(3,3)  V2=ones(3,3)  I1=ones(3,3)  I2=ones(3,3)  nHarmo=1  Measurements=None
  LIGNE_400_Kv_MATEUR_MORNAGUIA_CN_129996167_225000_CN_129996179_225000 : powerlib/Elements/Distributed Parameters Line  Phases=3  Frequency=50  Resistance=[0.01273 0.3864]  Inductance="[0.9337e-3  4.1264e-3]"  Capacitance=[12.74e-9 7.751e-9]  Length=49.4203  x1=[8.73114913702011e-11 380000 380000;314.159265358979 314.159265358979 314.159265358979;-0.177670123217348 0.415246442777429 -1.15554988401747]  x2=[1.26090477118469e-09 381852.398472139 381852.398472139;314.159265358979 314.159265358979 314.159265358979;-1.41941675517191 0.415007521738739 -1.15578880505616]  x3=[1.07663708898761e-11 1405.24743813465 1405.24743813466;314.159265358979 314.159265358979 314.159265358979;-2.70558821102223 0.316110507002444 -1.25468581979246]  x4=[8.62234243168895e-12 1405.96374414071 1405.9637441407;314.159265358979 314.159265358979 314.159265358979;0.245769282942371 0.405640215255436 -1.16515611153945]  x5=0.000565541566995742  V1=ones(3,3)  V2=ones(3,3)  I1=ones(3,3)  I2=ones(3,3)  nHarmo=1  Measurements=None
  L_{93263381,101404944,111375420,125504235,129996167,129996179,173531194,173534564,178328237,178494278,179549833,180611326,180615776,189193646,224416644,224417135,226848748,242398869} (18 alike) : powerlib/Elements/Three-Phase Series RLC Load  LConnTagsString=A|B|C  Configuration=Y (grounded)  NominalVoltage=225000  Vabc=[1e3 1e3 1e3]  Vabcp=[1e3 1e3 1e3]  NominalFrequency=50  UnbalancedPower=off  ActivePower=100000  InductivePower=100  CapacitivePower=100  Pabc=[10e3 9e3 11e3]  QLabc=[100 90 110]  QCabc=[100 90 110]  Pabcp=[10e3 9e3 11e3]  QLabcp=[100 90 110]  QCabcp=[100 90 110]  Measurements=None  LoadType=constant PQ
  L_{28943745,106469430,111375430,130775787,131220525,174150822,178326515,178543491,178547287,178549814,189193656,198577383,201812735,202286224,206389818,206449367,207339172,215133456,242384114,242390602,242392536,252371715,253586233,322419513} (24 alike) : powerlib/Elements/Three-Phase Series RLC Load  LConnTagsString=A|B|C  Configuration=Y (grounded)  NominalVoltage=150000  Vabc=[1e3 1e3 1e3]  Vabcp=[1e3 1e3 1e3]  NominalFrequency=50  UnbalancedPower=off  ActivePower=100000  InductivePower=100  CapacitivePower=100  Pabc=[10e3 9e3 11e3]  QLabc=[100 90 110]  QCabc=[100 90 110]  Pabcp=[10e3 9e3 11e3]  QLabcp=[100 90 110]  QCabcp=[100 90 110]  Measurements=None  LoadType=constant PQ
  Ligne_150_KV_Feriana_Mdhilla_CN_252371715_150000_CN_206449367_150000 : powerlib/Elements/Distributed Parameters Line  Phases=3  Frequency=50  Resistance=[0.01273 0.3864]  Inductance="[0.9337e-3  4.1264e-3]"  Capacitance=[12.74e-9 7.751e-9]  Length=82.1088  x1=[8.73114913702011e-11 380000 380000;314.159265358979 314.159265358979 314.159265358979;-0.177670123217348 0.415246442777429 -1.15554988401747]  x2=[1.26090477118469e-09 381852.398472139 381852.398472139;314.159265358979 314.159265358979 314.159265358979;-1.41941675517191 0.415007521738739 -1.15578880505616]  x3=[1.07663708898761e-11 1405.24743813465 1405.24743813466;314.159265358979 314.159265358979 314.159265358979;-2.70558821102223 0.316110507002444 -1.25468581979246]  x4=[8.62234243168895e-12 1405.96374414071 1405.9637441407;314.159265358979 314.159265358979 314.159265358979;0.245769282942371 0.405640215255436 -1.16515611153945]  x5=0.000565541566995742  V1=ones(3,3)  V2=ones(3,3)  I1=ones(3,3)  I2=ones(3,3)  nHarmo=1  Measurements=None
  T_101404944__POSTE_225_90_MNIHLA_1 : powerlib/Elements/Three-Phase Transformer (Two Windings)  Winding1Connection=Yg  Winding2Connection=Yg  CoreType=Three single-phase transformers  SetSaturation=off  Hysteresis=off  DataFile='hysteresis'  SetInitialFlux=off  Measurements=None  UNITS=pu  NominalPower=[ 250e6 , 50 ]  Winding1=[225000,0.002,0.08]  Winding2=[225000,0.002,0.08]  Rm=2000  Lm=50  L0=0.5  Saturation=[ 0,0 ; 0.0024,1.2 ; 1.0,1.52 ]  InitialFluxes=[ 0.8 , -0.8 , 0.7 ]  MoreParameters=off  BreakLoop=off  DataType=off  TransfoNumber=1
  T_106469430__POSTE_BOUFICHA : powerlib/Elements/Three-Phase Transformer (Two Windings)  Winding1Connection=Yg  Winding2Connection=Yg  CoreType=Three single-phase transformers  SetSaturation=off  Hysteresis=off  DataFile='hysteresis'  SetInitialFlux=off  Measurements=None  UNITS=pu  NominalPower=[ 250e6 , 50 ]  Winding1=[225000,0.002,0.08]  Winding2=[150000,0.002,0.08]  Rm=2000  Lm=50  L0=0.5  Saturation=[ 0,0 ; 0.0024,1.2 ; 1.0,1.52 ]  InitialFluxes=[ 0.8 , -0.8 , 0.7 ]  MoreParameters=off  BreakLoop=off  DataType=off  TransfoNumber=1
  T_111375420__POSTE_SOUSSE : powerlib/Elements/Three-Phase Transformer (Two Windings)  Winding1Connection=Yg  Winding2Connection=Yg  CoreType=Three single-phase transformers  SetSaturation=off  Hysteresis=off  DataFile='hysteresis'  SetInitialFlux=off  Measurements=None  UNITS=pu  NominalPower=[ 250e6 , 50 ]  Winding1=[225000,0.002,0.08]  Winding2=[225000,0.002,0.08]  Rm=2000  Lm=50  L0=0.5  Saturation=[ 0,0 ; 0.0024,1.2 ; 1.0,1.52 ]  InitialFluxes=[ 0.8 , -0.8 , 0.7 ]  MoreParameters=off  BreakLoop=off  DataType=off  TransfoNumber=1
  T_111375430__ : powerlib/Elements/Three-Phase Transformer (Two Windings)  Winding1Connection=Yg  Winding2Connection=Yg  CoreType=Three single-phase transformers  SetSaturation=off  Hysteresis=off  DataFile='hysteresis'  SetInitialFlux=off  Measurements=None  UNITS=pu  NominalPower=[ 250e6 , 50 ]  Winding1=[150000,0.002,0.08]  Winding2=[150000,0.002,0.08]  Rm=2000  Lm=50  L0=0.5  Saturation=[ 0,0 ; 0.0024,1.2 ; 1.0,1.52 ]  InitialFluxes=[ 0.8 , -0.8 , 0.7 ]  MoreParameters=off  BreakLoop=off  DataType=off  TransfoNumber=1
  T_125504235_225000_POSTE_NAASEN : powerlib/Elements/Three-Phase Transformer (Two Windings)  Winding1Connection=Yg  Winding2Connection=Yg  CoreType=Three single-phase transformers  SetSaturation=off  Hysteresis=off  DataFile='hysteresis'  SetInitialFlux=off  Measurements=None  UNITS=pu  NominalPower=[ 250e6 , 50 ]  Winding1=[225000,0.002,0.08]  Winding2=[225000,0.002,0.08]  Rm=2000  Lm=50  L0=0.5  Saturation=[ 0,0 ; 0.0024,1.2 ; 1.0,1.52 ]  InitialFluxes=[ 0.8 , -0.8 , 0.7 ]  MoreParameters=off  BreakLoop=off  DataType=off  TransfoNumber=1
  T_129996167__ : powerlib/Elements/Three-Phase Transformer (Two Windings)  Winding1Connection=Yg  Winding2Connection=Yg  CoreType=Three single-phase transformers  SetSaturation=off  Hysteresis=off  DataFile='hysteresis'  SetInitialFlux=off  Measurements=None  UNITS=pu  NominalPower=[ 250e6 , 50 ]  Winding1=[225000,0.002,0.08]  Winding2=[225000,0.002,0.08]  Rm=2000  Lm=50  L0=0.5  Saturation=[ 0,0 ; 0.0024,1.2 ; 1.0,1.52 ]  InitialFluxes=[ 0.8 , -0.8 , 0.7 ]  MoreParameters=off  BreakLoop=off  DataType=off  TransfoNumber=1
  T_129996179__POSTE_MATEUR : powerlib/Elements/Three-Phase Transformer (Two Windings)  Winding1Connection=Yg  Winding2Connection=Yg  CoreType=Three single-phase transformers  SetSaturation=off  Hysteresis=off  DataFile='hysteresis'  SetInitialFlux=off  Measurements=None  UNITS=pu  NominalPower=[ 250e6 , 50 ]  Winding1=[225000,0.002,0.08]  Winding2=[225000,0.002,0.08]  Rm=2000  Lm=50  L0=0.5  Saturation=[ 0,0 ; 0.0024,1.2 ; 1.0,1.52 ]  InitialFluxes=[ 0.8 , -0.8 , 0.7 ]  MoreParameters=off  BreakLoop=off  DataType=off  TransfoNumber=1
  T_130775787__POSTE_MSAKEN : powerlib/Elements/Three-Phase Transformer (Two Windings)  Winding1Connection=Yg  Winding2Connection=Yg  CoreType=Three single-phase transformers  SetSaturation=off  Hysteresis=off  DataFile='hysteresis'  SetInitialFlux=off  Measurements=None  UNITS=pu  NominalPower=[ 250e6 , 50 ]  Winding1=[150000,0.002,0.08]  Winding2=[150000,0.002,0.08]  Rm=2000  Lm=50  L0=0.5  Saturation=[ 0,0 ; 0.0024,1.2 ; 1.0,1.52 ]  InitialFluxes=[ 0.8 , -0.8 , 0.7 ]  MoreParameters=off  BreakLoop=off  DataType=off  TransfoNumber=1
  T_131220525__Poste__Enfidha_Sud : powerlib/Elements/Three-Phase Transformer (Two Windings)  Winding1Connection=Yg  Winding2Connection=Yg  CoreType=Three single-phase transformers  SetSaturation=off  Hysteresis=off  DataFile='hysteresis'  SetInitialFlux=off  Measurements=None  UNITS=pu  NominalPower=[ 250e6 , 50 ]  Winding1=[150000,0.002,0.08]  Winding2=[150000,0.002,0.08]  Rm=2000  Lm=50  L0=0.5  Saturation=[ 0,0 ; 0.0024,1.2 ; 1.0,1.52 ]  InitialFluxes=[ 0.8 , -0.8 , 0.7 ]  MoreParameters=off  BreakLoop=off  DataType=off  TransfoNumber=1
  T_173531194__POSTE_BIR_MCHARGA : powerlib/Elements/Three-Phase Transformer (Two Windings)  Winding1Connection=Yg  Winding2Connection=Yg  CoreType=Three single-phase transformers  SetSaturation=off  Hysteresis=off  DataFile='hysteresis'  SetInitialFlux=off  Measurements=None  UNITS=pu  NominalPower=[ 250e6 , 50 ]  Winding1=[225000,0.002,0.08]  Winding2=[225000,0.002,0.08]  Rm=2000  Lm=50  L0=0.5  Saturation=[ 0,0 ; 0.0024,1.2 ; 1.0,1.52 ]  InitialFluxes=[ 0.8 , -0.8 , 0.7 ]  MoreParameters=off  BreakLoop=off  DataType=off  TransfoNumber=1
  T_173534564__POSTE_JENDOUBA : powerlib/Elements/Three-Phase Transformer (Two Windings)  Winding1Connection=Yg  Winding2Connection=Yg  CoreType=Three single-phase transformers  SetSaturation=off  Hysteresis=off  DataFile='hysteresis'  SetInitialFlux=off  Measurements=None  UNITS=pu  NominalPower=[ 250e6 , 50 ]  Winding1=[225000,0.002,0.08]  Winding2=[225000,0.002,0.08]  Rm=2000  Lm=50  L0=0.5  Saturation=[ 0,0 ; 0.0024,1.2 ; 1.0,1.52 ]  InitialFluxes=[ 0.8 , -0.8 , 0.7 ]  MoreParameters=off  BreakLoop=off  DataType=off  TransfoNumber=1
  T_174150822__POSTE_LESSOUDA : powerlib/Elements/Three-Phase Transformer (Two Windings)  Winding1Connection=Yg  Winding2Connection=Yg  CoreType=Three single-phase transformers  SetSaturation=off  Hysteresis=off  DataFile='hysteresis'  SetInitialFlux=off  Measurements=None  UNITS=pu  NominalPower=[ 250e6 , 50 ]  Winding1=[150000,0.002,0.08]  Winding2=[150000,0.002,0.08]  Rm=2000  Lm=50  L0=0.5  Saturation=[ 0,0 ; 0.0024,1.2 ; 1.0,1.52 ]  InitialFluxes=[ 0.8 , -0.8 , 0.7 ]  MoreParameters=off  BreakLoop=off  DataType=off  TransfoNumber=1
  T_178326515__POSTE_MOKNINE : powerlib/Elements/Three-Phase Transformer (Two Windings)  Winding1Connection=Yg  Winding2Connection=Yg  CoreType=Three single-phase transformers  SetSaturation=off  Hysteresis=off  DataFile='hysteresis'  SetInitialFlux=off  Measurements=None  UNITS=pu  NominalPower=[ 250e6 , 50 ]  Winding1=[225000,0.002,0.08]  Winding2=[150000,0.002,0.08]  Rm=2000  Lm=50  L0=0.5  Saturation=[ 0,0 ; 0.0024,1.2 ; 1.0,1.52 ]  InitialFluxes=[ 0.8 , -0.8 , 0.7 ]  MoreParameters=off  BreakLoop=off  DataType=off  TransfoNumber=1
  T_178328237__POSTE_SIDI_MANSOUR : powerlib/Elements/Three-Phase Transformer (Two Windings)  Winding1Connection=Yg  Winding2Connection=Yg  CoreType=Three single-phase transformers  SetSaturation=off  Hysteresis=off  DataFile='hysteresis'  SetInitialFlux=off  Measurements=None  UNITS=pu  NominalPower=[ 250e6 , 50 ]  Winding1=[225000,0.002,0.08]  Winding2=[225000,0.002,0.08]  Rm=2000  Lm=50  L0=0.5  Saturation=[ 0,0 ; 0.0024,1.2 ; 1.0,1.52 ]  InitialFluxes=[ 0.8 , -0.8 , 0.7 ]  MoreParameters=off  BreakLoop=off  DataType=off  TransfoNumber=1
  T_178494278__POSTE_MENZEL_JEMIL : powerlib/Elements/Three-Phase Transformer (Two Windings)  Winding1Connection=Yg  Winding2Connection=Yg  CoreType=Three single-phase transformers  SetSaturation=off  Hysteresis=off  DataFile='hysteresis'  SetInitialFlux=off  Measurements=None  UNITS=pu  NominalPower=[ 250e6 , 50 ]  Winding1=[225000,0.002,0.08]  Winding2=[225000,0.002,0.08]  Rm=2000  Lm=50  L0=0.5  Saturation=[ 0,0 ; 0.0024,1.2 ; 1.0,1.52 ]  InitialFluxes=[ 0.8 , -0.8 , 0.7 ]  MoreParameters=off  BreakLoop=off  DataType=off  TransfoNumber=1
  T_178543491__POSTE_GREMDA : powerlib/Elements/Three-Phase Transformer (Two Windings)  Winding1Connection=Yg  Winding2Connection=Yg  CoreType=Three single-phase transformers  SetSaturation=off  Hysteresis=off  DataFile='hysteresis'  SetInitialFlux=off  Measurements=None  UNITS=pu  NominalPower=[ 250e6 , 50 ]  Winding1=[150000,0.002,0.08]  Winding2=[150000,0.002,0.08]  Rm=2000  Lm=50  L0=0.5  Saturation=[ 0,0 ; 0.0024,1.2 ; 1.0,1.52 ]  InitialFluxes=[ 0.8 , -0.8 , 0.7 ]  MoreParameters=off  BreakLoop=off  DataType=off  TransfoNumber=1
  T_178547287__POSTE_THYNA : powerlib/Elements/Three-Phase Transformer (Two Windings)  Winding1Connection=Yg  Winding2Connection=Yg  CoreType=Three single-phase transformers  SetSaturation=off  Hysteresis=off  DataFile='hysteresis'  SetInitialFlux=off  Measurements=None  UNITS=pu  NominalPower=[ 250e6 , 50 ]  Winding1=[150000,0.002,0.08]  Winding2=[150000,0.002,0.08]  Rm=2000  Lm=50  L0=0.5  Saturation=[ 0,0 ; 0.0024,1.2 ; 1.0,1.52 ]  InitialFluxes=[ 0.8 , -0.8 , 0.7 ]  MoreParameters=off  BreakLoop=off  DataType=off  TransfoNumber=1
  T_178549814__POSTE_ELJEM : powerlib/Elements/Three-Phase Transformer (Two Windings)  Winding1Connection=Yg  Winding2Connection=Yg  CoreType=Three single-phase transformers  SetSaturation=off  Hysteresis=off  DataFile='hysteresis'  SetInitialFlux=off  Measurements=None  UNITS=pu  NominalPower=[ 250e6 , 50 ]  Winding1=[150000,0.002,0.08]  Winding2=[150000,0.002,0.08]  Rm=2000  Lm=50  L0=0.5  Saturation=[ 0,0 ; 0.0024,1.2 ; 1.0,1.52 ]  InitialFluxes=[ 0.8 , -0.8 , 0.7 ]  MoreParameters=off  BreakLoop=off  DataType=off  TransfoNumber=1
  T_179549833__POSTE_TAJEROUINE_225_KV : powerlib/Elements/Three-Phase Transformer (Two Windings)  Winding1Connection=Yg  Winding2Connection=Yg  CoreType=Three single-phase transformers  SetSaturation=off  Hysteresis=off  DataFile='hysteresis'  SetInitialFlux=off  Measurements=None  UNITS=pu  NominalPower=[ 250e6 , 50 ]  Winding1=[225000,0.002,0.08]  Winding2=[225000,0.002,0.08]  Rm=2000  Lm=50  L0=0.5  Saturation=[ 0,0 ; 0.0024,1.2 ; 1.0,1.52 ]  InitialFluxes=[ 0.8 , -0.8 , 0.7 ]  MoreParameters=off  BreakLoop=off  DataType=off  TransfoNumber=1
  T_180611326__POSTE_MEDENINE : powerlib/Elements/Three-Phase Transformer (Two Windings)  Winding1Connection=Yg  Winding2Connection=Yg  CoreType=Three single-phase transformers  SetSaturation=off  Hysteresis=off  DataFile='hysteresis'  SetInitialFlux=off  Measurements=None  UNITS=pu  NominalPower=[ 250e6 , 50 ]  Winding1=[225000,0.002,0.08]  Winding2=[225000,0.002,0.08]  Rm=2000  Lm=50  L0=0.5  Saturation=[ 0,0 ; 0.0024,1.2 ; 1.0,1.52 ]  InitialFluxes=[ 0.8 , -0.8 , 0.7 ]  MoreParameters=off  BreakLoop=off  DataType=off  TransfoNumber=1
  T_180615776__POSTE_TATAOUINE : powerlib/Elements/Three-Phase Transformer (Two Windings)  Winding1Connection=Yg  Winding2Connection=Yg  CoreType=Three single-phase transformers  SetSaturation=off  Hysteresis=off  DataFile='hysteresis'  SetInitialFlux=off  Measurements=None  UNITS=pu  NominalPower=[ 250e6 , 50 ]  Winding1=[225000,0.002,0.08]  Winding2=[225000,0.002,0.08]  Rm=2000  Lm=50  L0=0.5  Saturation=[ 0,0 ; 0.0024,1.2 ; 1.0,1.52 ]  InitialFluxes=[ 0.8 , -0.8 , 0.7 ]  MoreParameters=off  BreakLoop=off  DataType=off  TransfoNumber=1
  T_189193646__POSTE_BOUCHEMMA : powerlib/Elements/Three-Phase Transformer (Two Windings)  Winding1Connection=Yg  Winding2Connection=Yg  CoreType=Three single-phase transformers  SetSaturation=off  Hysteresis=off  DataFile='hysteresis'  SetInitialFlux=off  Measurements=None  UNITS=pu  NominalPower=[ 250e6 , 50 ]  Winding1=[225000,0.002,0.08]  Winding2=[225000,0.002,0.08]  Rm=2000  Lm=50  L0=0.5  Saturation=[ 0,0 ; 0.0024,1.2 ; 1.0,1.52 ]  InitialFluxes=[ 0.8 , -0.8 , 0.7 ]  MoreParameters=off  BreakLoop=off  DataType=off  TransfoNumber=1
  T_189193656__ : powerlib/Elements/Three-Phase Transformer (Two Windings)  Winding1Connection=Yg  Winding2Connection=Yg  CoreType=Three single-phase transformers  SetSaturation=off  Hysteresis=off  DataFile='hysteresis'  SetInitialFlux=off  Measurements=None  UNITS=pu  NominalPower=[ 250e6 , 50 ]  Winding1=[225000,0.002,0.08]  Winding2=[150000,0.002,0.08]  Rm=2000  Lm=50  L0=0.5  Saturation=[ 0,0 ; 0.0024,1.2 ; 1.0,1.52 ]  InitialFluxes=[ 0.8 , -0.8 , 0.7 ]  MoreParameters=off  BreakLoop=off  DataType=off  TransfoNumber=1
  T_198577383__POSTE_ROBBANA : powerlib/Elements/Three-Phase Transformer (Two Windings)  Winding1Connection=Yg  Winding2Connection=Yg  CoreType=Three single-phase transformers  SetSaturation=off  Hysteresis=off  DataFile='hysteresis'  SetInitialFlux=off  Measurements=None  UNITS=pu  NominalPower=[ 250e6 , 50 ]  Winding1=[150000,0.002,0.08]  Winding2=[150000,0.002,0.08]  Rm=2000  Lm=50  L0=0.5  Saturation=[ 0,0 ; 0.0024,1.2 ; 1.0,1.52 ]  InitialFluxes=[ 0.8 , -0.8 , 0.7 ]  MoreParameters=off  BreakLoop=off  DataType=off  TransfoNumber=1
  T_201812735__POSTE_MEKNASSY : powerlib/Elements/Three-Phase Transformer (Two Windings)  Winding1Connection=Yg  Winding2Connection=Yg  CoreType=Three single-phase transformers  SetSaturation=off  Hysteresis=off  DataFile='hysteresis'  SetInitialFlux=off  Measurements=None  UNITS=pu  NominalPower=[ 250e6 , 50 ]  Winding1=[225000,0.002,0.08]  Winding2=[150000,0.002,0.08]  Rm=2000  Lm=50  L0=0.5  Saturation=[ 0,0 ; 0.0024,1.2 ; 1.0,1.52 ]  InitialFluxes=[ 0.8 , -0.8 , 0.7 ]  MoreParameters=off  BreakLoop=off  DataType=off  TransfoNumber=1
  T_202286224__POSTE_SKHIRA : powerlib/Elements/Three-Phase Transformer (Two Windings)  Winding1Connection=Yg  Winding2Connection=Yg  CoreType=Three single-phase transformers  SetSaturation=off  Hysteresis=off  DataFile='hysteresis'  SetInitialFlux=off  Measurements=None  UNITS=pu  NominalPower=[ 250e6 , 50 ]  Winding1=[150000,0.002,0.08]  Winding2=[150000,0.002,0.08]  Rm=2000  Lm=50  L0=0.5  Saturation=[ 0,0 ; 0.0024,1.2 ; 1.0,1.52 ]  InitialFluxes=[ 0.8 , -0.8 , 0.7 ]  MoreParameters=off  BreakLoop=off  DataType=off  TransfoNumber=1
  T_206389818__POSTE_METLAOUI : powerlib/Elements/Three-Phase Transformer (Two Windings)  Winding1Connection=Yg  Winding2Connection=Yg  CoreType=Three single-phase transformers  SetSaturation=off  Hysteresis=off  DataFile='hysteresis'  SetInitialFlux=off  Measurements=None  UNITS=pu  NominalPower=[ 250e6 , 50 ]  Winding1=[150000,0.002,0.08]  Winding2=[150000,0.002,0.08]  Rm=2000  Lm=50  L0=0.5  Saturation=[ 0,0 ; 0.0024,1.2 ; 1.0,1.52 ]  InitialFluxes=[ 0.8 , -0.8 , 0.7 ]  MoreParameters=off  BreakLoop=off  DataType=off  TransfoNumber=1
  T_206449367_150000_POSTE_DE_MDHILLA : powerlib/Elements/Three-Phase Transformer (Two Windings)  Winding1Connection=Yg  Winding2Connection=Yg  CoreType=Three single-phase transformers  SetSaturation=off  Hysteresis=off  DataFile='hysteresis'  SetInitialFlux=off  Measurements=None  UNITS=pu  NominalPower=[ 250e6 , 50 ]  Winding1=[150000,0.002,0.08]  Winding2=[150000,0.002,0.08]  Rm=2000  Lm=50  L0=0.5  Saturation=[ 0,0 ; 0.0024,1.2 ; 1.0,1.52 ]  InitialFluxes=[ 0.8 , -0.8 , 0.7 ]  MoreParameters=off  BreakLoop=off  DataType=off  TransfoNumber=1
  T_207339172__POSTE_TOZEUR : powerlib/Elements/Three-Phase Transformer (Two Windings)  Winding1Connection=Yg  Winding2Connection=Yg  CoreType=Three single-phase transformers  SetSaturation=off  Hysteresis=off  DataFile='hysteresis'  SetInitialFlux=off  Measurements=None  UNITS=pu  NominalPower=[ 250e6 , 50 ]  Winding1=[150000,0.002,0.08]  Winding2=[150000,0.002,0.08]  Rm=2000  Lm=50  L0=0.5  Saturation=[ 0,0 ; 0.0024,1.2 ; 1.0,1.52 ]  InitialFluxes=[ 0.8 , -0.8 , 0.7 ]  MoreParameters=off  BreakLoop=off  DataType=off  TransfoNumber=1
  T_215133456__POSTE_MIDOUN : powerlib/Elements/Three-Phase Transformer (Two Windings)  Winding1Connection=Yg  Winding2Connection=Yg  CoreType=Three single-phase transformers  SetSaturation=off  Hysteresis=off  DataFile='hysteresis'  SetInitialFlux=off  Measurements=None  UNITS=pu  NominalPower=[ 250e6 , 50 ]  Winding1=[150000,0.002,0.08]  Winding2=[150000,0.002,0.08]  Rm=2000  Lm=50  L0=0.5  Saturation=[ 0,0 ; 0.0024,1.2 ; 1.0,1.52 ]  InitialFluxes=[ 0.8 , -0.8 , 0.7 ]  MoreParameters=off  BreakLoop=off  DataType=off  TransfoNumber=1
  T_224416644__POSTE_OUESLATIA : powerlib/Elements/Three-Phase Transformer (Two Windings)  Winding1Connection=Yg  Winding2Connection=Yg  CoreType=Three single-phase transformers  SetSaturation=off  Hysteresis=off  DataFile='hysteresis'  SetInitialFlux=off  Measurements=None  UNITS=pu  NominalPower=[ 250e6 , 50 ]  Winding1=[225000,0.002,0.08]  Winding2=[225000,0.002,0.08]  Rm=2000  Lm=50  L0=0.5  Saturation=[ 0,0 ; 0.0024,1.2 ; 1.0,1.52 ]  InitialFluxes=[ 0.8 , -0.8 , 0.7 ]  MoreParameters=off  BreakLoop=off  DataType=off  TransfoNumber=1
  T_224417135__POSTE_HAJEB_LAYOUN : powerlib/Elements/Three-Phase Transformer (Two Windings)  Winding1Connection=Yg  Winding2Connection=Yg  CoreType=Three single-phase transformers  SetSaturation=off  Hysteresis=off  DataFile='hysteresis'  SetInitialFlux=off  Measurements=None  UNITS=pu  NominalPower=[ 250e6 , 50 ]  Winding1=[225000,0.002,0.08]  Winding2=[225000,0.002,0.08]  Rm=2000  Lm=50  L0=0.5  Saturation=[ 0,0 ; 0.0024,1.2 ; 1.0,1.52 ]  InitialFluxes=[ 0.8 , -0.8 , 0.7 ]  MoreParameters=off  BreakLoop=off  DataType=off  TransfoNumber=1
  T_226848748__ : powerlib/Elements/Three-Phase Transformer (Two Windings)  Winding1Connection=Yg  Winding2Connection=Yg  CoreType=Three single-phase transformers  SetSaturation=off  Hysteresis=off  DataFile='hysteresis'  SetInitialFlux=off  Measurements=None  UNITS=pu  NominalPower=[ 250e6 , 50 ]  Winding1=[225000,0.002,0.08]  Winding2=[225000,0.002,0.08]  Rm=2000  Lm=50  L0=0.5  Saturation=[ 0,0 ; 0.0024,1.2 ; 1.0,1.52 ]  InitialFluxes=[ 0.8 , -0.8 , 0.7 ]  MoreParameters=off  BreakLoop=off  DataType=off  TransfoNumber=1
  T_242384114__POSTE_ZARZIS : powerlib/Elements/Three-Phase Transformer (Two Windings)  Winding1Connection=Yg  Winding2Connection=Yg  CoreType=Three single-phase transformers  SetSaturation=off  Hysteresis=off  DataFile='hysteresis'  SetInitialFlux=off  Measurements=None  UNITS=pu  NominalPower=[ 250e6 , 50 ]  Winding1=[150000,0.002,0.08]  Winding2=[150000,0.002,0.08]  Rm=2000  Lm=50  L0=0.5  Saturation=[ 0,0 ; 0.0024,1.2 ; 1.0,1.52 ]  InitialFluxes=[ 0.8 , -0.8 , 0.7 ]  MoreParameters=off  BreakLoop=off  DataType=off  TransfoNumber=1
  T_242390602__POSTE_DE_GHANNOUCH : powerlib/Elements/Three-Phase Transformer (Two Windings)  Winding1Connection=Yg  Winding2Connection=Yg  CoreType=Three single-phase transformers  SetSaturation=off  Hysteresis=off  DataFile='hysteresis'  SetInitialFlux=off  Measurements=None  UNITS=pu  NominalPower=[ 250e6 , 50 ]  Winding1=[150000,0.002,0.08]  Winding2=[150000,0.002,0.08]  Rm=2000  Lm=50  L0=0.5  Saturation=[ 0,0 ; 0.0024,1.2 ; 1.0,1.52 ]  InitialFluxes=[ 0.8 , -0.8 , 0.7 ]  MoreParameters=off  BreakLoop=off  DataType=off  TransfoNumber=1
  T_242392536__POSTE_GABES_SUD : powerlib/Elements/Three-Phase Transformer (Two Windings)  Winding1Connection=Yg  Winding2Connection=Yg  CoreType=Three single-phase transformers  SetSaturation=off  Hysteresis=off  DataFile='hysteresis'  SetInitialFlux=off  Measurements=None  UNITS=pu  NominalPower=[ 250e6 , 50 ]  Winding1=[150000,0.002,0.08]  Winding2=[150000,0.002,0.08]  Rm=2000  Lm=50  L0=0.5  Saturation=[ 0,0 ; 0.0024,1.2 ; 1.0,1.52 ]  InitialFluxes=[ 0.8 , -0.8 , 0.7 ]  MoreParameters=off  BreakLoop=off  DataType=off  TransfoNumber=1
  T_242398869__POSTE_KAIROUAN : powerlib/Elements/Three-Phase Transformer (Two Windings)  Winding1Connection=Yg  Winding2Connection=Yg  CoreType=Three single-phase transformers  SetSaturation=off  Hysteresis=off  DataFile='hysteresis'  SetInitialFlux=off  Measurements=None  UNITS=pu  NominalPower=[ 250e6 , 50 ]  Winding1=[225000,0.002,0.08]  Winding2=[225000,0.002,0.08]  Rm=2000  Lm=50  L0=0.5  Saturation=[ 0,0 ; 0.0024,1.2 ; 1.0,1.52 ]  InitialFluxes=[ 0.8 , -0.8 , 0.7 ]  MoreParameters=off  BreakLoop=off  DataType=off  TransfoNumber=1
  T_252371715__POSTE_FERIANA : powerlib/Elements/Three-Phase Transformer (Two Windings)  Winding1Connection=Yg  Winding2Connection=Yg  CoreType=Three single-phase transformers  SetSaturation=off  Hysteresis=off  DataFile='hysteresis'  SetInitialFlux=off  Measurements=None  UNITS=pu  NominalPower=[ 250e6 , 50 ]  Winding1=[150000,0.002,0.08]  Winding2=[150000,0.002,0.08]  Rm=2000  Lm=50  L0=0.5  Saturation=[ 0,0 ; 0.0024,1.2 ; 1.0,1.52 ]  InitialFluxes=[ 0.8 , -0.8 , 0.7 ]  MoreParameters=off  BreakLoop=off  DataType=off  TransfoNumber=1
  T_253586233__POSTE_DE_KEBILI : powerlib/Elements/Three-Phase Transformer (Two Windings)  Winding1Connection=Yg  Winding2Connection=Yg  CoreType=Three single-phase transformers  SetSaturation=off  Hysteresis=off  DataFile='hysteresis'  SetInitialFlux=off  Measurements=None  UNITS=pu  NominalPower=[ 250e6 , 50 ]  Winding1=[150000,0.002,0.08]  Winding2=[150000,0.002,0.08]  Rm=2000  Lm=50  L0=0.5  Saturation=[ 0,0 ; 0.0024,1.2 ; 1.0,1.52 ]  InitialFluxes=[ 0.8 , -0.8 , 0.7 ]  MoreParameters=off  BreakLoop=off  DataType=off  TransfoNumber=1
  T_28943745__POSTE_MSAKEN_NORD : powerlib/Elements/Three-Phase Transformer (Two Windings)  Winding1Connection=Yg  Winding2Connection=Yg  CoreType=Three single-phase transformers  SetSaturation=off  Hysteresis=off  DataFile='hysteresis'  SetInitialFlux=off  Measurements=None  UNITS=pu  NominalPower=[ 250e6 , 50 ]  Winding1=[225000,0.002,0.08]  Winding2=[150000,0.002,0.08]  Rm=2000  Lm=50  L0=0.5  Saturation=[ 0,0 ; 0.0024,1.2 ; 1.0,1.52 ]  InitialFluxes=[ 0.8 , -0.8 , 0.7 ]  MoreParameters=off  BreakLoop=off  DataType=off  TransfoNumber=1
  T_322419513__POSTE_DE_LA_CIMENTERIE_DE_GABES : powerlib/Elements/Three-Phase Transformer (Two Windings)  Winding1Connection=Yg  Winding2Connection=Yg  CoreType=Three single-phase transformers  SetSaturation=off  Hysteresis=off  DataFile='hysteresis'  SetInitialFlux=off  Measurements=None  UNITS=pu  NominalPower=[ 250e6 , 50 ]  Winding1=[150000,0.002,0.08]  Winding2=[150000,0.002,0.08]  Rm=2000  Lm=50  L0=0.5  Saturation=[ 0,0 ; 0.0024,1.2 ; 1.0,1.52 ]  InitialFluxes=[ 0.8 , -0.8 , 0.7 ]  MoreParameters=off  BreakLoop=off  DataType=off  TransfoNumber=1
  T_93263381__POSTE_RADES : powerlib/Elements/Three-Phase Transformer (Two Windings)  Winding1Connection=Yg  Winding2Connection=Yg  CoreType=Three single-phase transformers  SetSaturation=off  Hysteresis=off  DataFile='hysteresis'  SetInitialFlux=off  Measurements=None  UNITS=pu  NominalPower=[ 250e6 , 50 ]  Winding1=[225000,0.002,0.08]  Winding2=[225000,0.002,0.08]  Rm=2000  Lm=50  L0=0.5  Saturation=[ 0,0 ; 0.0024,1.2 ; 1.0,1.52 ]  InitialFluxes=[ 0.8 , -0.8 , 0.7 ]  MoreParameters=off  BreakLoop=off  DataType=off  TransfoNumber=1
  _CN_101404944_225000_CN_93164455_225000 : powerlib/Elements/Distributed Parameters Line  Phases=3  Frequency=50  Resistance=[0.01273 0.3864]  Inductance="[0.9337e-3  4.1264e-3]"  Capacitance=[12.74e-9 7.751e-9]  Length=25.554  x1=[8.73114913702011e-11 380000 380000;314.159265358979 314.159265358979 314.159265358979;-0.177670123217348 0.415246442777429 -1.15554988401747]  x2=[1.26090477118469e-09 381852.398472139 381852.398472139;314.159265358979 314.159265358979 314.159265358979;-1.41941675517191 0.415007521738739 -1.15578880505616]  x3=[1.07663708898761e-11 1405.24743813465 1405.24743813466;314.159265358979 314.159265358979 314.159265358979;-2.70558821102223 0.316110507002444 -1.25468581979246]  x4=[8.62234243168895e-12 1405.96374414071 1405.9637441407;314.159265358979 314.159265358979 314.159265358979;0.245769282942371 0.405640215255436 -1.16515611153945]  x5=0.000565541566995742  V1=ones(3,3)  V2=ones(3,3)  I1=ones(3,3)  I2=ones(3,3)  nHarmo=1  Measurements=None
  _CN_129996167_225000_CN_101404944_225000 : powerlib/Elements/Distributed Parameters Line  Phases=3  Frequency=50  Resistance=[0.01273 0.3864]  Inductance="[0.9337e-3  4.1264e-3]"  Capacitance=[12.74e-9 7.751e-9]  Length=56.598  x1=[8.73114913702011e-11 380000 380000;314.159265358979 314.159265358979 314.159265358979;-0.177670123217348 0.415246442777429 -1.15554988401747]  x2=[1.26090477118469e-09 381852.398472139 381852.398472139;314.159265358979 314.159265358979 314.159265358979;-1.41941675517191 0.415007521738739 -1.15578880505616]  x3=[1.07663708898761e-11 1405.24743813465 1405.24743813466;314.159265358979 314.159265358979 314.159265358979;-2.70558821102223 0.316110507002444 -1.25468581979246]  x4=[8.62234243168895e-12 1405.96374414071 1405.9637441407;314.159265358979 314.159265358979 314.159265358979;0.245769282942371 0.405640215255436 -1.16515611153945]  x5=0.000565541566995742  V1=ones(3,3)  V2=ones(3,3)  I1=ones(3,3)  I2=ones(3,3)  nHarmo=1  Measurements=None
  _CN_129996167_225000_CN_173531194_225000 : powerlib/Elements/Distributed Parameters Line  Phases=3  Frequency=50  Resistance=[0.01273 0.3864]  Inductance="[0.9337e-3  4.1264e-3]"  Capacitance=[12.74e-9 7.751e-9]  Length=119.0291  x1=[8.73114913702011e-11 380000 380000;314.159265358979 314.159265358979 314.159265358979;-0.177670123217348 0.415246442777429 -1.15554988401747]  x2=[1.26090477118469e-09 381852.398472139 381852.398472139;314.159265358979 314.159265358979 314.159265358979;-1.41941675517191 0.415007521738739 -1.15578880505616]  x3=[1.07663708898761e-11 1405.24743813465 1405.24743813466;314.159265358979 314.159265358979 314.159265358979;-2.70558821102223 0.316110507002444 -1.25468581979246]  x4=[8.62234243168895e-12 1405.96374414071 1405.9637441407;314.159265358979 314.159265358979 314.159265358979;0.245769282942371 0.405640215255436 -1.16515611153945]  x5=0.000565541566995742  V1=ones(3,3)  V2=ones(3,3)  I1=ones(3,3)  I2=ones(3,3)  nHarmo=1  Measurements=None
  _CN_178328237_225000_CN_189193646_225000 : powerlib/Elements/Distributed Parameters Line  Phases=3  Frequency=50  Resistance=[0.01273 0.3864]  Inductance="[0.9337e-3  4.1264e-3]"  Capacitance=[12.74e-9 7.751e-9]  Length=72.0148  x1=[8.73114913702011e-11 380000 380000;314.159265358979 314.159265358979 314.159265358979;-0.177670123217348 0.415246442777429 -1.15554988401747]  x2=[1.26090477118469e-09 381852.398472139 381852.398472139;314.159265358979 314.159265358979 314.159265358979;-1.41941675517191 0.415007521738739 -1.15578880505616]  x3=[1.07663708898761e-11 1405.24743813465 1405.24743813466;314.159265358979 314.159265358979 314.159265358979;-2.70558821102223 0.316110507002444 -1.25468581979246]  x4=[8.62234243168895e-12 1405.96374414071 1405.9637441407;314.159265358979 314.159265358979 314.159265358979;0.245769282942371 0.405640215255436 -1.16515611153945]  x5=0.000565541566995742  V1=ones(3,3)  V2=ones(3,3)  I1=ones(3,3)  I2=ones(3,3)  nHarmo=1  Measurements=None
  _CN_189193646_225000_CN_180611326_225000 : powerlib/Elements/Distributed Parameters Line  Phases=3  Frequency=50  Resistance=[0.01273 0.3864]  Inductance="[0.9337e-3  4.1264e-3]"  Capacitance=[12.74e-9 7.751e-9]  Length=10.2256  x1=[8.73114913702011e-11 380000 380000;314.159265358979 314.159265358979 314.159265358979;-0.177670123217348 0.415246442777429 -1.15554988401747]  x2=[1.26090477118469e-09 381852.398472139 381852.398472139;314.159265358979 314.159265358979 314.159265358979;-1.41941675517191 0.415007521738739 -1.15578880505616]  x3=[1.07663708898761e-11 1405.24743813465 1405.24743813466;314.159265358979 314.159265358979 314.159265358979;-2.70558821102223 0.316110507002444 -1.25468581979246]  x4=[8.62234243168895e-12 1405.96374414071 1405.9637441407;314.159265358979 314.159265358979 314.159265358979;0.245769282942371 0.405640215255436 -1.16515611153945]  x5=0.000565541566995742  V1=ones(3,3)  V2=ones(3,3)  I1=ones(3,3)  I2=ones(3,3)  nHarmo=1  Measurements=None
  _CN_189193646_225000_CN_189193656_225000 : powerlib/Elements/Distributed Parameters Line  Phases=3  Frequency=50  Resistance=[0.01273 0.3864]  Inductance="[0.9337e-3  4.1264e-3]"  Capacitance=[12.74e-9 7.751e-9]  Length=0.87897  x1=[8.73114913702011e-11 380000 380000;314.159265358979 314.159265358979 314.159265358979;-0.177670123217348 0.415246442777429 -1.15554988401747]  x2=[1.26090477118469e-09 381852.398472139 381852.398472139;314.159265358979 314.159265358979 314.159265358979;-1.41941675517191 0.415007521738739 -1.15578880505616]  x3=[1.07663708898761e-11 1405.24743813465 1405.24743813466;314.159265358979 314.159265358979 314.159265358979;-2.70558821102223 0.316110507002444 -1.25468581979246]  x4=[8.62234243168895e-12 1405.96374414071 1405.9637441407;314.159265358979 314.159265358979 314.159265358979;0.245769282942371 0.405640215255436 -1.16515611153945]  x5=0.000565541566995742  V1=ones(3,3)  V2=ones(3,3)  I1=ones(3,3)  I2=ones(3,3)  nHarmo=1  Measurements=None
  _CN_189193656_150000_CN_206449367_150000 : powerlib/Elements/Distributed Parameters Line  Phases=3  Frequency=50  Resistance=[0.01273 0.3864]  Inductance="[0.9337e-3  4.1264e-3]"  Capacitance=[12.74e-9 7.751e-9]  Length=59.7218  x1=[8.73114913702011e-11 380000 380000;314.159265358979 314.159265358979 314.159265358979;-0.177670123217348 0.415246442777429 -1.15554988401747]  x2=[1.26090477118469e-09 381852.398472139 381852.398472139;314.159265358979 314.159265358979 314.159265358979;-1.41941675517191 0.415007521738739 -1.15578880505616]  x3=[1.07663708898761e-11 1405.24743813465 1405.24743813466;314.159265358979 314.159265358979 314.159265358979;-2.70558821102223 0.316110507002444 -1.25468581979246]  x4=[8.62234243168895e-12 1405.96374414071 1405.9637441407;314.159265358979 314.159265358979 314.159265358979;0.245769282942371 0.405640215255436 -1.16515611153945]  x5=0.000565541566995742  V1=ones(3,3)  V2=ones(3,3)  I1=ones(3,3)  I2=ones(3,3)  nHarmo=1  Measurements=None
  _CN_189193656_150000_CN_242390602_150000 : powerlib/Elements/Distributed Parameters Line  Phases=3  Frequency=50  Resistance=[0.01273 0.3864]  Inductance="[0.9337e-3  4.1264e-3]"  Capacitance=[12.74e-9 7.751e-9]  Length=4.6625  x1=[8.73114913702011e-11 380000 380000;314.159265358979 314.159265358979 314.159265358979;-0.177670123217348 0.415246442777429 -1.15554988401747]  x2=[1.26090477118469e-09 381852.398472139 381852.398472139;314.159265358979 314.159265358979 314.159265358979;-1.41941675517191 0.415007521738739 -1.15578880505616]  x3=[1.07663708898761e-11 1405.24743813465 1405.24743813466;314.159265358979 314.159265358979 314.159265358979;-2.70558821102223 0.316110507002444 -1.25468581979246]  x4=[8.62234243168895e-12 1405.96374414071 1405.9637441407;314.159265358979 314.159265358979 314.159265358979;0.245769282942371 0.405640215255436 -1.16515611153945]  x5=0.000565541566995742  V1=ones(3,3)  V2=ones(3,3)  I1=ones(3,3)  I2=ones(3,3)  nHarmo=1  Measurements=None
  _CN_252371715_150000_CN_206389818_150000 : powerlib/Elements/Distributed Parameters Line  Phases=3  Frequency=50  Resistance=[0.01273 0.3864]  Inductance="[0.9337e-3  4.1264e-3]"  Capacitance=[12.74e-9 7.751e-9]  Length=72.8627  x1=[8.73114913702011e-11 380000 380000;314.159265358979 314.159265358979 314.159265358979;-0.177670123217348 0.415246442777429 -1.15554988401747]  x2=[1.26090477118469e-09 381852.398472139 381852.398472139;314.159265358979 314.159265358979 314.159265358979;-1.41941675517191 0.415007521738739 -1.15578880505616]  x3=[1.07663708898761e-11 1405.24743813465 1405.24743813466;314.159265358979 314.159265358979 314.159265358979;-2.70558821102223 0.316110507002444 -1.25468581979246]  x4=[8.62234243168895e-12 1405.96374414071 1405.9637441407;314.159265358979 314.159265358979 314.159265358979;0.245769282942371 0.405640215255436 -1.16515611153945]  x5=0.000565541566995742  V1=ones(3,3)  V2=ones(3,3)  I1=ones(3,3)  I2=ones(3,3)  nHarmo=1  Measurements=None
  _CN_28943745_225000_CN_111375420_225000 : powerlib/Elements/Distributed Parameters Line  Phases=3  Frequency=50  Resistance=[0.01273 0.3864]  Inductance="[0.9337e-3  4.1264e-3]"  Capacitance=[12.74e-9 7.751e-9]  Length=15.4681  x1=[8.73114913702011e-11 380000 380000;314.159265358979 314.159265358979 314.159265358979;-0.177670123217348 0.415246442777429 -1.15554988401747]  x2=[1.26090477118469e-09 381852.398472139 381852.398472139;314.159265358979 314.159265358979 314.159265358979;-1.41941675517191 0.415007521738739 -1.15578880505616]  x3=[1.07663708898761e-11 1405.24743813465 1405.24743813466;314.159265358979 314.159265358979 314.159265358979;-2.70558821102223 0.316110507002444 -1.25468581979246]  x4=[8.62234243168895e-12 1405.96374414071 1405.9637441407;314.159265358979 314.159265358979 314.159265358979;0.245769282942371 0.405640215255436 -1.16515611153945]  x5=0.000565541566995742  V1=ones(3,3)  V2=ones(3,3)  I1=ones(3,3)  I2=ones(3,3)  nHarmo=1  Measurements=None
  _CN_28943745_225000_CN_224416644_225000 : powerlib/Elements/Distributed Parameters Line  Phases=3  Frequency=50  Resistance=[0.01273 0.3864]  Inductance="[0.9337e-3  4.1264e-3]"  Capacitance=[12.74e-9 7.751e-9]  Length=88.9841  x1=[8.73114913702011e-11 380000 380000;314.159265358979 314.159265358979 314.159265358979;-0.177670123217348 0.415246442777429 -1.15554988401747]  x2=[1.26090477118469e-09 381852.398472139 381852.398472139;314.159265358979 314.159265358979 314.159265358979;-1.41941675517191 0.415007521738739 -1.15578880505616]  x3=[1.07663708898761e-11 1405.24743813465 1405.24743813466;314.159265358979 314.159265358979 314.159265358979;-2.70558821102223 0.316110507002444 -1.25468581979246]  x4=[8.62234243168895e-12 1405.96374414071 1405.9637441407;314.159265358979 314.159265358979 314.159265358979;0.245769282942371 0.405640215255436 -1.16515611153945]  x5=0.000565541566995742  V1=ones(3,3)  V2=ones(3,3)  I1=ones(3,3)  I2=ones(3,3)  nHarmo=1  Measurements=None
  bus1 : powerlib/Measurements/Load Flow Bus  LConnTagsString=a  Phases=single  Connectors=on one side  ID=bus1  Vbase=150000  Vref=1  Vangle=0  VLF=1  VLFb=1  VLFc=1  angleLF=0  angleLFb=0  angleLFc=0
      settings: AttributesFormatString=|
      | %<ID>
      | %<Vbase>V
      | %<VLF>pu
      | %<angleLF>deg.
      | %<Name>
  bus10 : powerlib/Measurements/Load Flow Bus  LConnTagsString=a  Phases=single  Connectors=on one side  ID=bus10  Vbase=150000  Vref=1  Vangle=0  VLF=1  VLFb=1  VLFc=1  angleLF=0  angleLFb=0  angleLFc=0
      settings: AttributesFormatString=|
      | %<ID>
      | %<Vbase>V
      | %<VLF>pu
      | %<angleLF>deg.
      | %<Name>
  bus11 : powerlib/Measurements/Load Flow Bus  LConnTagsString=a  Phases=single  Connectors=on one side  ID=bus11  Vbase=150000  Vref=1  Vangle=0  VLF=1  VLFb=1  VLFc=1  angleLF=0  angleLFb=0  angleLFc=0
      settings: AttributesFormatString=|
      | %<ID>
      | %<Vbase>V
      | %<VLF>pu
      | %<angleLF>deg.
      | %<Name>
  bus12 : powerlib/Measurements/Load Flow Bus  LConnTagsString=a  Phases=single  Connectors=on one side  ID=bus12  Vbase=150000  Vref=1  Vangle=0  VLF=1  VLFb=1  VLFc=1  angleLF=0  angleLFb=0  angleLFc=0
      settings: AttributesFormatString=|
      | %<ID>
      | %<Vbase>V
      | %<VLF>pu
      | %<angleLF>deg.
      | %<Name>
  bus13 : powerlib/Measurements/Load Flow Bus  LConnTagsString=a  Phases=single  Connectors=on one side  ID=bus13  Vbase=150000  Vref=1  Vangle=0  VLF=1  VLFb=1  VLFc=1  angleLF=0  angleLFb=0  angleLFc=0
      settings: AttributesFormatString=|
      | %<ID>
      | %<Vbase>V
      | %<VLF>pu
      | %<angleLF>deg.
      | %<Name>
  bus14 : powerlib/Measurements/Load Flow Bus  LConnTagsString=a  Phases=single  Connectors=on one side  ID=bus14  Vbase=150000  Vref=1  Vangle=0  VLF=1  VLFb=1  VLFc=1  angleLF=0  angleLFb=0  angleLFc=0
      settings: AttributesFormatString=|
      | %<ID>
      | %<Vbase>V
      | %<VLF>pu
      | %<angleLF>deg.
      | %<Name>
  bus15 : powerlib/Measurements/Load Flow Bus  LConnTagsString=a  Phases=single  Connectors=on one side  ID=bus15  Vbase=150000  Vref=1  Vangle=0  VLF=1  VLFb=1  VLFc=1  angleLF=0  angleLFb=0  angleLFc=0
      settings: AttributesFormatString=|
      | %<ID>
      | %<Vbase>V
      | %<VLF>pu
      | %<angleLF>deg.
      | %<Name>
  bus16 : powerlib/Measurements/Load Flow Bus  LConnTagsString=a  Phases=single  Connectors=on one side  ID=bus16  Vbase=150000  Vref=1  Vangle=0  VLF=1  VLFb=1  VLFc=1  angleLF=0  angleLFb=0  angleLFc=0
      settings: AttributesFormatString=|
      | %<ID>
      | %<Vbase>V
      | %<VLF>pu
      | %<angleLF>deg.
      | %<Name>
  bus17 : powerlib/Measurements/Load Flow Bus  LConnTagsString=a  Phases=single  Connectors=on one side  ID=bus17  Vbase=150000  Vref=1  Vangle=0  VLF=1  VLFb=1  VLFc=1  angleLF=0  angleLFb=0  angleLFc=0
      settings: AttributesFormatString=|
      | %<ID>
      | %<Vbase>V
      | %<VLF>pu
      | %<angleLF>deg.
      | %<Name>
  bus18 : powerlib/Measurements/Load Flow Bus  LConnTagsString=a  Phases=single  Connectors=on one side  ID=bus18  Vbase=150000  Vref=1  Vangle=0  VLF=1  VLFb=1  VLFc=1  angleLF=0  angleLFb=0  angleLFc=0
      settings: AttributesFormatString=|
      | %<ID>
      | %<Vbase>V
      | %<VLF>pu
      | %<angleLF>deg.
      | %<Name>
  bus19 : powerlib/Measurements/Load Flow Bus  LConnTagsString=a  Phases=single  Connectors=on one side  ID=bus19  Vbase=150000  Vref=1  Vangle=0  VLF=1  VLFb=1  VLFc=1  angleLF=0  angleLFb=0  angleLFc=0
      settings: AttributesFormatString=|
      | %<ID>
      | %<Vbase>V
      | %<VLF>pu
      | %<angleLF>deg.
      | %<Name>
  bus2 : powerlib/Measurements/Load Flow Bus  LConnTagsString=a  Phases=single  Connectors=on one side  ID=bus2  Vbase=150000  Vref=1  Vangle=0  VLF=1  VLFb=1  VLFc=1  angleLF=0  angleLFb=0  angleLFc=0
      settings: AttributesFormatString=|
      | %<ID>
      | %<Vbase>V
      | %<VLF>pu
      | %<angleLF>deg.
      | %<Name>
  bus20 : powerlib/Measurements/Load Flow Bus  LConnTagsString=a  Phases=single  Connectors=on one side  ID=bus20  Vbase=150000  Vref=1  Vangle=0  VLF=1  VLFb=1  VLFc=1  angleLF=0  angleLFb=0  angleLFc=0
      settings: AttributesFormatString=|
      | %<ID>
      | %<Vbase>V
      | %<VLF>pu
      | %<angleLF>deg.
      | %<Name>
  bus21 : powerlib/Measurements/Load Flow Bus  LConnTagsString=a  Phases=single  Connectors=on one side  ID=bus21  Vbase=150000  Vref=1  Vangle=0  VLF=1  VLFb=1  VLFc=1  angleLF=0  angleLFb=0  angleLFc=0
      settings: AttributesFormatString=|
      | %<ID>
      | %<Vbase>V
      | %<VLF>pu
      | %<angleLF>deg.
      | %<Name>
  bus22 : powerlib/Measurements/Load Flow Bus  LConnTagsString=a  Phases=single  Connectors=on one side  ID=bus22  Vbase=150000  Vref=1  Vangle=0  VLF=1  VLFb=1  VLFc=1  angleLF=0  angleLFb=0  angleLFc=0
      settings: AttributesFormatString=|
      | %<ID>
      | %<Vbase>V
      | %<VLF>pu
      | %<angleLF>deg.
      | %<Name>
  bus23 : powerlib/Measurements/Load Flow Bus  LConnTagsString=a  Phases=single  Connectors=on one side  ID=bus23  Vbase=150000  Vref=1  Vangle=0  VLF=1  VLFb=1  VLFc=1  angleLF=0  angleLFb=0  angleLFc=0
      settings: AttributesFormatString=|
      | %<ID>
      | %<Vbase>V
      | %<VLF>pu
      | %<angleLF>deg.
      | %<Name>
  bus24 : powerlib/Measurements/Load Flow Bus  LConnTagsString=a  Phases=single  Connectors=on one side  ID=bus24  Vbase=150000  Vref=1  Vangle=0  VLF=1  VLFb=1  VLFc=1  angleLF=0  angleLFb=0  angleLFc=0
      settings: AttributesFormatString=|
      | %<ID>
      | %<Vbase>V
      | %<VLF>pu
      | %<angleLF>deg.
      | %<Name>
  bus25 : powerlib/Measurements/Load Flow Bus  LConnTagsString=a  Phases=single  Connectors=on one side  ID=bus25  Vbase=225000  Vref=1  Vangle=0  VLF=1  VLFb=1  VLFc=1  angleLF=0  angleLFb=0  angleLFc=0
      settings: AttributesFormatString=|
      | %<ID>
      | %<Vbase>V
      | %<VLF>pu
      | %<angleLF>deg.
      | %<Name>
  bus26 : powerlib/Measurements/Load Flow Bus  LConnTagsString=a  Phases=single  Connectors=on one side  ID=bus26  Vbase=225000  Vref=1  Vangle=0  VLF=1  VLFb=1  VLFc=1  angleLF=0  angleLFb=0  angleLFc=0
      settings: AttributesFormatString=|
      | %<ID>
      | %<Vbase>V
      | %<VLF>pu
      | %<angleLF>deg.
      | %<Name>
  bus27 : powerlib/Measurements/Load Flow Bus  LConnTagsString=a  Phases=single  Connectors=on one side  ID=bus27  Vbase=225000  Vref=1  Vangle=0  VLF=1  VLFb=1  VLFc=1  angleLF=0  angleLFb=0  angleLFc=0
      settings: AttributesFormatString=|
      | %<ID>
      | %<Vbase>V
      | %<VLF>pu
      | %<angleLF>deg.
      | %<Name>
  bus28 : powerlib/Measurements/Load Flow Bus  LConnTagsString=a  Phases=single  Connectors=on one side  ID=bus28  Vbase=225000  Vref=1  Vangle=0  VLF=1  VLFb=1  VLFc=1  angleLF=0  angleLFb=0  angleLFc=0
      settings: AttributesFormatString=|
      | %<ID>
      | %<Vbase>V
      | %<VLF>pu
      | %<angleLF>deg.
      | %<Name>
  bus29 : powerlib/Measurements/Load Flow Bus  LConnTagsString=a  Phases=single  Connectors=on one side  ID=bus29  Vbase=225000  Vref=1  Vangle=0  VLF=1  VLFb=1  VLFc=1  angleLF=0  angleLFb=0  angleLFc=0
      settings: AttributesFormatString=|
      | %<ID>
      | %<Vbase>V
      | %<VLF>pu
      | %<angleLF>deg.
      | %<Name>
  bus3 : powerlib/Measurements/Load Flow Bus  LConnTagsString=a  Phases=single  Connectors=on one side  ID=bus3  Vbase=150000  Vref=1  Vangle=0  VLF=1  VLFb=1  VLFc=1  angleLF=0  angleLFb=0  angleLFc=0
      settings: AttributesFormatString=|
      | %<ID>
      | %<Vbase>V
      | %<VLF>pu
      | %<angleLF>deg.
      | %<Name>
  bus30 : powerlib/Measurements/Load Flow Bus  LConnTagsString=a  Phases=single  Connectors=on one side  ID=bus30  Vbase=225000  Vref=1  Vangle=0  VLF=1  VLFb=1  VLFc=1  angleLF=0  angleLFb=0  angleLFc=0
      settings: AttributesFormatString=|
      | %<ID>
      | %<Vbase>V
      | %<VLF>pu
      | %<angleLF>deg.
      | %<Name>
  bus31 : powerlib/Measurements/Load Flow Bus  LConnTagsString=a  Phases=single  Connectors=on one side  ID=bus31  Vbase=225000  Vref=1  Vangle=0  VLF=1  VLFb=1  VLFc=1  angleLF=0  angleLFb=0  angleLFc=0
      settings: AttributesFormatString=|
      | %<ID>
      | %<Vbase>V
      | %<VLF>pu
      | %<angleLF>deg.
      | %<Name>
  bus32 : powerlib/Measurements/Load Flow Bus  LConnTagsString=a  Phases=single  Connectors=on one side  ID=bus32  Vbase=225000  Vref=1  Vangle=0  VLF=1  VLFb=1  VLFc=1  angleLF=0  angleLFb=0  angleLFc=0
      settings: AttributesFormatString=|
      | %<ID>
      | %<Vbase>V
      | %<VLF>pu
      | %<angleLF>deg.
      | %<Name>
  bus33 : powerlib/Measurements/Load Flow Bus  LConnTagsString=a  Phases=single  Connectors=on one side  ID=bus33  Vbase=225000  Vref=1  Vangle=0  VLF=1  VLFb=1  VLFc=1  angleLF=0  angleLFb=0  angleLFc=0
      settings: AttributesFormatString=|
      | %<ID>
      | %<Vbase>V
      | %<VLF>pu
      | %<angleLF>deg.
      | %<Name>
  bus34 : powerlib/Measurements/Load Flow Bus  LConnTagsString=a  Phases=single  Connectors=on one side  ID=bus34  Vbase=225000  Vref=1  Vangle=0  VLF=1  VLFb=1  VLFc=1  angleLF=0  angleLFb=0  angleLFc=0
      settings: AttributesFormatString=|
      | %<ID>
      | %<Vbase>V
      | %<VLF>pu
      | %<angleLF>deg.
      | %<Name>
  bus35 : powerlib/Measurements/Load Flow Bus  LConnTagsString=a  Phases=single  Connectors=on one side  ID=bus35  Vbase=225000  Vref=1  Vangle=0  VLF=1  VLFb=1  VLFc=1  angleLF=0  angleLFb=0  angleLFc=0
      settings: AttributesFormatString=|
      | %<ID>
      | %<Vbase>V
      | %<VLF>pu
      | %<angleLF>deg.
      | %<Name>
  bus36 : powerlib/Measurements/Load Flow Bus  LConnTagsString=a  Phases=single  Connectors=on one side  ID=bus36  Vbase=225000  Vref=1  Vangle=0  VLF=1  VLFb=1  VLFc=1  angleLF=0  angleLFb=0  angleLFc=0
      settings: AttributesFormatString=|
      | %<ID>
      | %<Vbase>V
      | %<VLF>pu
      | %<angleLF>deg.
      | %<Name>
  bus37 : powerlib/Measurements/Load Flow Bus  LConnTagsString=a  Phases=single  Connectors=on one side  ID=bus37  Vbase=225000  Vref=1  Vangle=0  VLF=1  VLFb=1  VLFc=1  angleLF=0  angleLFb=0  angleLFc=0
      settings: AttributesFormatString=|
      | %<ID>
      | %<Vbase>V
      | %<VLF>pu
      | %<angleLF>deg.
      | %<Name>
  bus38 : powerlib/Measurements/Load Flow Bus  LConnTagsString=a  Phases=single  Connectors=on one side  ID=bus38  Vbase=225000  Vref=1  Vangle=0  VLF=1  VLFb=1  VLFc=1  angleLF=0  angleLFb=0  angleLFc=0
      settings: AttributesFormatString=|
      | %<ID>
      | %<Vbase>V
      | %<VLF>pu
      | %<angleLF>deg.
      | %<Name>
  bus39 : powerlib/Measurements/Load Flow Bus  LConnTagsString=a  Phases=single  Connectors=on one side  ID=bus39  Vbase=225000  Vref=1  Vangle=0  VLF=1  VLFb=1  VLFc=1  angleLF=0  angleLFb=0  angleLFc=0
      settings: AttributesFormatString=|
      | %<ID>
      | %<Vbase>V
      | %<VLF>pu
      | %<angleLF>deg.
      | %<Name>
  bus4 : powerlib/Measurements/Load Flow Bus  LConnTagsString=a  Phases=single  Connectors=on one side  ID=bus4  Vbase=150000  Vref=1  Vangle=0  VLF=1  VLFb=1  VLFc=1  angleLF=0  angleLFb=0  angleLFc=0
      settings: AttributesFormatString=|
      | %<ID>
      | %<Vbase>V
      | %<VLF>pu
      | %<angleLF>deg.
      | %<Name>
  bus40 : powerlib/Measurements/Load Flow Bus  LConnTagsString=a  Phases=single  Connectors=on one side  ID=bus40  Vbase=225000  Vref=1  Vangle=0  VLF=1  VLFb=1  VLFc=1  angleLF=0  angleLFb=0  angleLFc=0
      settings: AttributesFormatString=|
      | %<ID>
      | %<Vbase>V
      | %<VLF>pu
      | %<angleLF>deg.
      | %<Name>
  bus41 : powerlib/Measurements/Load Flow Bus  LConnTagsString=a  Phases=single  Connectors=on one side  ID=bus41  Vbase=225000  Vref=1  Vangle=0  VLF=1  VLFb=1  VLFc=1  angleLF=0  angleLFb=0  angleLFc=0
      settings: AttributesFormatString=|
      | %<ID>
      | %<Vbase>V
      | %<VLF>pu
      | %<angleLF>deg.
      | %<Name>
  bus42 : powerlib/Measurements/Load Flow Bus  LConnTagsString=a  Phases=single  Connectors=on one side  ID=bus42  Vbase=225000  Vref=1  Vangle=0  VLF=1  VLFb=1  VLFc=1  angleLF=0  angleLFb=0  angleLFc=0
      settings: AttributesFormatString=|
      | %<ID>
      | %<Vbase>V
      | %<VLF>pu
      | %<angleLF>deg.
      | %<Name>
  bus43 : powerlib/Measurements/Load Flow Bus  LConnTagsString=a  Phases=single  Connectors=on one side  ID=bus43  Vbase=225000  Vref=1  Vangle=0  VLF=1  VLFb=1  VLFc=1  angleLF=0  angleLFb=0  angleLFc=0
      settings: AttributesFormatString=|
      | %<ID>
      | %<Vbase>V
      | %<VLF>pu
      | %<angleLF>deg.
      | %<Name>
  bus44 : powerlib/Measurements/Load Flow Bus  LConnTagsString=a  Phases=single  Connectors=on one side  ID=bus44  Vbase=225000  Vref=1  Vangle=0  VLF=1  VLFb=1  VLFc=1  angleLF=0  angleLFb=0  angleLFc=0
      settings: AttributesFormatString=|
      | %<ID>
      | %<Vbase>V
      | %<VLF>pu
      | %<angleLF>deg.
      | %<Name>
  bus45 : powerlib/Measurements/Load Flow Bus  LConnTagsString=a  Phases=single  Connectors=on one side  ID=bus45  Vbase=225000  Vref=1  Vangle=0  VLF=1  VLFb=1  VLFc=1  angleLF=0  angleLFb=0  angleLFc=0
      settings: AttributesFormatString=|
      | %<ID>
      | %<Vbase>V
      | %<VLF>pu
      | %<angleLF>deg.
      | %<Name>
  bus46 : powerlib/Measurements/Load Flow Bus  LConnTagsString=a  Phases=single  Connectors=on one side  ID=bus46  Vbase=225000  Vref=1  Vangle=0  VLF=1  VLFb=1  VLFc=1  angleLF=0  angleLFb=0  angleLFc=0
      settings: AttributesFormatString=|
      | %<ID>
      | %<Vbase>V
      | %<VLF>pu
      | %<angleLF>deg.
      | %<Name>
  bus47 : powerlib/Measurements/Load Flow Bus  LConnTagsString=a  Phases=single  Connectors=on one side  ID=bus47  Vbase=225000  Vref=1  Vangle=0  VLF=1  VLFb=1  VLFc=1  angleLF=0  angleLFb=0  angleLFc=0
      settings: AttributesFormatString=|
      | %<ID>
      | %<Vbase>V
      | %<VLF>pu
      | %<angleLF>deg.
      | %<Name>
  bus48 : powerlib/Measurements/Load Flow Bus  LConnTagsString=a  Phases=single  Connectors=on one side  ID=bus48  Vbase=225000  Vref=1  Vangle=0  VLF=1  VLFb=1  VLFc=1  angleLF=0  angleLFb=0  angleLFc=0
      settings: AttributesFormatString=|
      | %<ID>
      | %<Vbase>V
      | %<VLF>pu
      | %<angleLF>deg.
      | %<Name>
  bus49 : powerlib/Measurements/Load Flow Bus  LConnTagsString=a  Phases=single  Connectors=on one side  ID=bus49  Vbase=150000  Vref=1  Vangle=0  VLF=1  VLFb=1  VLFc=1  angleLF=0  angleLFb=0  angleLFc=0
      settings: AttributesFormatString=|
      | %<ID>
      | %<Vbase>V
      | %<VLF>pu
      | %<angleLF>deg.
      | %<Name>
  bus5 : powerlib/Measurements/Load Flow Bus  LConnTagsString=a  Phases=single  Connectors=on one side  ID=bus5  Vbase=150000  Vref=1  Vangle=0  VLF=1  VLFb=1  VLFc=1  angleLF=0  angleLFb=0  angleLFc=0
      settings: AttributesFormatString=|
      | %<ID>
      | %<Vbase>V
      | %<VLF>pu
      | %<angleLF>deg.
      | %<Name>
  bus50 : powerlib/Measurements/Load Flow Bus  LConnTagsString=a  Phases=single  Connectors=on one side  ID=bus50  Vbase=150000  Vref=1  Vangle=0  VLF=1  VLFb=1  VLFc=1  angleLF=0  angleLFb=0  angleLFc=0
      settings: AttributesFormatString=|
      | %<ID>
      | %<Vbase>V
      | %<VLF>pu
      | %<angleLF>deg.
      | %<Name>
  bus51 : powerlib/Measurements/Load Flow Bus  LConnTagsString=a  Phases=single  Connectors=on one side  ID=bus51  Vbase=150000  Vref=1  Vangle=0  VLF=1  VLFb=1  VLFc=1  angleLF=0  angleLFb=0  angleLFc=0
      settings: AttributesFormatString=|
      | %<ID>
      | %<Vbase>V
      | %<VLF>pu
      | %<angleLF>deg.
      | %<Name>
  bus52 : powerlib/Measurements/Load Flow Bus  LConnTagsString=a  Phases=single  Connectors=on one side  ID=bus52  Vbase=150000  Vref=1  Vangle=0  VLF=1  VLFb=1  VLFc=1  angleLF=0  angleLFb=0  angleLFc=0
      settings: AttributesFormatString=|
      | %<ID>
      | %<Vbase>V
      | %<VLF>pu
      | %<angleLF>deg.
      | %<Name>
  bus53 : powerlib/Measurements/Load Flow Bus  LConnTagsString=a  Phases=single  Connectors=on one side  ID=bus53  Vbase=150000  Vref=1  Vangle=0  VLF=1  VLFb=1  VLFc=1  angleLF=0  angleLFb=0  angleLFc=0
      settings: AttributesFormatString=|
      | %<ID>
      | %<Vbase>V
      | %<VLF>pu
      | %<angleLF>deg.
      | %<Name>
  bus54 : powerlib/Measurements/Load Flow Bus  LConnTagsString=a  Phases=single  Connectors=on one side  ID=bus54  Vbase=150000  Vref=1  Vangle=0  VLF=1  VLFb=1  VLFc=1  angleLF=0  angleLFb=0  angleLFc=0
      settings: AttributesFormatString=|
      | %<ID>
      | %<Vbase>V
      | %<VLF>pu
      | %<angleLF>deg.
      | %<Name>
  bus55 : powerlib/Measurements/Load Flow Bus  LConnTagsString=a  Phases=single  Connectors=on one side  ID=bus55  Vbase=150000  Vref=1  Vangle=0  VLF=1  VLFb=1  VLFc=1  angleLF=0  angleLFb=0  angleLFc=0
      settings: AttributesFormatString=|
      | %<ID>
      | %<Vbase>V
      | %<VLF>pu
      | %<angleLF>deg.
      | %<Name>
  bus56 : powerlib/Measurements/Load Flow Bus  LConnTagsString=a  Phases=single  Connectors=on one side  ID=bus56  Vbase=150000  Vref=1  Vangle=0  VLF=1  VLFb=1  VLFc=1  angleLF=0  angleLFb=0  angleLFc=0
      settings: AttributesFormatString=|
      | %<ID>
      | %<Vbase>V
      | %<VLF>pu
      | %<angleLF>deg.
      | %<Name>
  bus57 : powerlib/Measurements/Load Flow Bus  LConnTagsString=a  Phases=single  Connectors=on one side  ID=bus57  Vbase=150000  Vref=1  Vangle=0  VLF=1  VLFb=1  VLFc=1  angleLF=0  angleLFb=0  angleLFc=0
      settings: AttributesFormatString=|
      | %<ID>
      | %<Vbase>V
      | %<VLF>pu
      | %<angleLF>deg.
      | %<Name>
  bus58 : powerlib/Measurements/Load Flow Bus  LConnTagsString=a  Phases=single  Connectors=on one side  ID=bus58  Vbase=150000  Vref=1  Vangle=0  VLF=1  VLFb=1  VLFc=1  angleLF=0  angleLFb=0  angleLFc=0
      settings: AttributesFormatString=|
      | %<ID>
      | %<Vbase>V
      | %<VLF>pu
      | %<angleLF>deg.
      | %<Name>
  bus59 : powerlib/Measurements/Load Flow Bus  LConnTagsString=a  Phases=single  Connectors=on one side  ID=bus59  Vbase=150000  Vref=1  Vangle=0  VLF=1  VLFb=1  VLFc=1  angleLF=0  angleLFb=0  angleLFc=0
      settings: AttributesFormatString=|
      | %<ID>
      | %<Vbase>V
      | %<VLF>pu
      | %<angleLF>deg.
      | %<Name>
  bus6 : powerlib/Measurements/Load Flow Bus  LConnTagsString=a  Phases=single  Connectors=on one side  ID=bus6  Vbase=150000  Vref=1  Vangle=0  VLF=1  VLFb=1  VLFc=1  angleLF=0  angleLFb=0  angleLFc=0
      settings: AttributesFormatString=|
      | %<ID>
      | %<Vbase>V
      | %<VLF>pu
      | %<angleLF>deg.
      | %<Name>
  bus60 : powerlib/Measurements/Load Flow Bus  LConnTagsString=a  Phases=single  Connectors=on one side  ID=bus60  Vbase=150000  Vref=1  Vangle=0  VLF=1  VLFb=1  VLFc=1  angleLF=0  angleLFb=0  angleLFc=0
      settings: AttributesFormatString=|
      | %<ID>
      | %<Vbase>V
      | %<VLF>pu
      | %<angleLF>deg.
      | %<Name>
  bus61 : powerlib/Measurements/Load Flow Bus  LConnTagsString=a  Phases=single  Connectors=on one side  ID=bus61  Vbase=150000  Vref=1  Vangle=0  VLF=1  VLFb=1  VLFc=1  angleLF=0  angleLFb=0  angleLFc=0
      settings: AttributesFormatString=|
      | %<ID>
      | %<Vbase>V
      | %<VLF>pu
      | %<angleLF>deg.
      | %<Name>
  bus62 : powerlib/Measurements/Load Flow Bus  LConnTagsString=a  Phases=single  Connectors=on one side  ID=bus62  Vbase=150000  Vref=1  Vangle=0  VLF=1  VLFb=1  VLFc=1  angleLF=0  angleLFb=0  angleLFc=0
      settings: AttributesFormatString=|
      | %<ID>
      | %<Vbase>V
      | %<VLF>pu
      | %<angleLF>deg.
      | %<Name>
  bus63 : powerlib/Measurements/Load Flow Bus  LConnTagsString=a  Phases=single  Connectors=on one side  ID=bus63  Vbase=150000  Vref=1  Vangle=0  VLF=1  VLFb=1  VLFc=1  angleLF=0  angleLFb=0  angleLFc=0
      settings: AttributesFormatString=|
      | %<ID>
      | %<Vbase>V
      | %<VLF>pu
      | %<angleLF>deg.
      | %<Name>
  bus64 : powerlib/Measurements/Load Flow Bus  LConnTagsString=a  Phases=single  Connectors=on one side  ID=bus64  Vbase=150000  Vref=1  Vangle=0  VLF=1  VLFb=1  VLFc=1  angleLF=0  angleLFb=0  angleLFc=0
      settings: AttributesFormatString=|
      | %<ID>
      | %<Vbase>V
      | %<VLF>pu
      | %<angleLF>deg.
      | %<Name>
  bus65 : powerlib/Measurements/Load Flow Bus  LConnTagsString=a  Phases=single  Connectors=on one side  ID=bus65  Vbase=150000  Vref=1  Vangle=0  VLF=1  VLFb=1  VLFc=1  angleLF=0  angleLFb=0  angleLFc=0
      settings: AttributesFormatString=|
      | %<ID>
      | %<Vbase>V
      | %<VLF>pu
      | %<angleLF>deg.
      | %<Name>
  bus66 : powerlib/Measurements/Load Flow Bus  LConnTagsString=a  Phases=single  Connectors=on one side  ID=bus66  Vbase=150000  Vref=1  Vangle=0  VLF=1  VLFb=1  VLFc=1  angleLF=0  angleLFb=0  angleLFc=0
      settings: AttributesFormatString=|
      | %<ID>
      | %<Vbase>V
      | %<VLF>pu
      | %<angleLF>deg.
      | %<Name>
  bus67 : powerlib/Measurements/Load Flow Bus  LConnTagsString=a  Phases=single  Connectors=on one side  ID=bus67  Vbase=150000  Vref=1  Vangle=0  VLF=1  VLFb=1  VLFc=1  angleLF=0  angleLFb=0  angleLFc=0
      settings: AttributesFormatString=|
      | %<ID>
      | %<Vbase>V
      | %<VLF>pu
      | %<angleLF>deg.
      | %<Name>
  bus68 : powerlib/Measurements/Load Flow Bus  LConnTagsString=a  Phases=single  Connectors=on one side  ID=bus68  Vbase=225000  Vref=1  Vangle=0  VLF=1  VLFb=1  VLFc=1  angleLF=0  angleLFb=0  angleLFc=0
      settings: AttributesFormatString=|
      | %<ID>
      | %<Vbase>V
      | %<VLF>pu
      | %<angleLF>deg.
      | %<Name>
  bus69 : powerlib/Measurements/Load Flow Bus  LConnTagsString=a  Phases=single  Connectors=on one side  ID=bus69  Vbase=225000  Vref=1  Vangle=0  VLF=1  VLFb=1  VLFc=1  angleLF=0  angleLFb=0  angleLFc=0
      settings: AttributesFormatString=|
      | %<ID>
      | %<Vbase>V
      | %<VLF>pu
      | %<angleLF>deg.
      | %<Name>
  bus7 : powerlib/Measurements/Load Flow Bus  LConnTagsString=a  Phases=single  Connectors=on one side  ID=bus7  Vbase=150000  Vref=1  Vangle=0  VLF=1  VLFb=1  VLFc=1  angleLF=0  angleLFb=0  angleLFc=0
      settings: AttributesFormatString=|
      | %<ID>
      | %<Vbase>V
      | %<VLF>pu
      | %<angleLF>deg.
      | %<Name>
  bus70 : powerlib/Measurements/Load Flow Bus  LConnTagsString=a  Phases=single  Connectors=on one side  ID=bus70  Vbase=225000  Vref=1  Vangle=0  VLF=1  VLFb=1  VLFc=1  angleLF=0  angleLFb=0  angleLFc=0
      settings: AttributesFormatString=|
      | %<ID>
      | %<Vbase>V
      | %<VLF>pu
      | %<angleLF>deg.
      | %<Name>
  bus71 : powerlib/Measurements/Load Flow Bus  LConnTagsString=a  Phases=single  Connectors=on one side  ID=bus71  Vbase=225000  Vref=1  Vangle=0  VLF=1  VLFb=1  VLFc=1  angleLF=0  angleLFb=0  angleLFc=0
      settings: AttributesFormatString=|
      | %<ID>
      | %<Vbase>V
      | %<VLF>pu
      | %<angleLF>deg.
      | %<Name>
  bus72 : powerlib/Measurements/Load Flow Bus  LConnTagsString=a  Phases=single  Connectors=on one side  ID=bus72  Vbase=225000  Vref=1  Vangle=0  VLF=1  VLFb=1  VLFc=1  angleLF=0  angleLFb=0  angleLFc=0
      settings: AttributesFormatString=|
      | %<ID>
      | %<Vbase>V
      | %<VLF>pu
      | %<angleLF>deg.
      | %<Name>
  bus73 : powerlib/Measurements/Load Flow Bus  LConnTagsString=a  Phases=single  Connectors=on one side  ID=bus73  Vbase=225000  Vref=1  Vangle=0  VLF=1  VLFb=1  VLFc=1  angleLF=0  angleLFb=0  angleLFc=0
      settings: AttributesFormatString=|
      | %<ID>
      | %<Vbase>V
      | %<VLF>pu
      | %<angleLF>deg.
      | %<Name>
  bus74 : powerlib/Measurements/Load Flow Bus  LConnTagsString=a  Phases=single  Connectors=on one side  ID=bus74  Vbase=225000  Vref=1  Vangle=0  VLF=1  VLFb=1  VLFc=1  angleLF=0  angleLFb=0  angleLFc=0
      settings: AttributesFormatString=|
      | %<ID>
      | %<Vbase>V
      | %<VLF>pu
      | %<angleLF>deg.
      | %<Name>
  bus75 : powerlib/Measurements/Load Flow Bus  LConnTagsString=a  Phases=single  Connectors=on one side  ID=bus75  Vbase=225000  Vref=1  Vangle=0  VLF=1  VLFb=1  VLFc=1  angleLF=0  angleLFb=0  angleLFc=0
      settings: AttributesFormatString=|
      | %<ID>
      | %<Vbase>V
      | %<VLF>pu
      | %<angleLF>deg.
      | %<Name>
  bus76 : powerlib/Measurements/Load Flow Bus  LConnTagsString=a  Phases=single  Connectors=on one side  ID=bus76  Vbase=225000  Vref=1  Vangle=0  VLF=1  VLFb=1  VLFc=1  angleLF=0  angleLFb=0  angleLFc=0
      settings: AttributesFormatString=|
      | %<ID>
      | %<Vbase>V
      | %<VLF>pu
      | %<angleLF>deg.
      | %<Name>
  bus77 : powerlib/Measurements/Load Flow Bus  LConnTagsString=a  Phases=single  Connectors=on one side  ID=bus77  Vbase=225000  Vref=1  Vangle=0  VLF=1  VLFb=1  VLFc=1  angleLF=0  angleLFb=0  angleLFc=0
      settings: AttributesFormatString=|
      | %<ID>
      | %<Vbase>V
      | %<VLF>pu
      | %<angleLF>deg.
      | %<Name>
  bus78 : powerlib/Measurements/Load Flow Bus  LConnTagsString=a  Phases=single  Connectors=on one side  ID=bus78  Vbase=225000  Vref=1  Vangle=0  VLF=1  VLFb=1  VLFc=1  angleLF=0  angleLFb=0  angleLFc=0
      settings: AttributesFormatString=|
      | %<ID>
      | %<Vbase>V
      | %<VLF>pu
      | %<angleLF>deg.
      | %<Name>
  bus79 : powerlib/Measurements/Load Flow Bus  LConnTagsString=a  Phases=single  Connectors=on one side  ID=bus79  Vbase=225000  Vref=1  Vangle=0  VLF=1  VLFb=1  VLFc=1  angleLF=0  angleLFb=0  angleLFc=0
      settings: AttributesFormatString=|
      | %<ID>
      | %<Vbase>V
      | %<VLF>pu
      | %<angleLF>deg.
      | %<Name>
  bus8 : powerlib/Measurements/Load Flow Bus  LConnTagsString=a  Phases=single  Connectors=on one side  ID=bus8  Vbase=150000  Vref=1  Vangle=0  VLF=1  VLFb=1  VLFc=1  angleLF=0  angleLFb=0  angleLFc=0
      settings: AttributesFormatString=|
      | %<ID>
      | %<Vbase>V
      | %<VLF>pu
      | %<angleLF>deg.
      | %<Name>
  bus80 : powerlib/Measurements/Load Flow Bus  LConnTagsString=a  Phases=single  Connectors=on one side  ID=bus80  Vbase=225000  Vref=1  Vangle=0  VLF=1  VLFb=1  VLFc=1  angleLF=0  angleLFb=0  angleLFc=0
      settings: AttributesFormatString=|
      | %<ID>
      | %<Vbase>V
      | %<VLF>pu
      | %<angleLF>deg.
      | %<Name>
  bus81 : powerlib/Measurements/Load Flow Bus  LConnTagsString=a  Phases=single  Connectors=on one side  ID=bus81  Vbase=225000  Vref=1  Vangle=0  VLF=1  VLFb=1  VLFc=1  angleLF=0  angleLFb=0  angleLFc=0
      settings: AttributesFormatString=|
      | %<ID>
      | %<Vbase>V
      | %<VLF>pu
      | %<angleLF>deg.
      | %<Name>
  bus82 : powerlib/Measurements/Load Flow Bus  LConnTagsString=a  Phases=single  Connectors=on one side  ID=bus82  Vbase=225000  Vref=1  Vangle=0  VLF=1  VLFb=1  VLFc=1  angleLF=0  angleLFb=0  angleLFc=0
      settings: AttributesFormatString=|
      | %<ID>
      | %<Vbase>V
      | %<VLF>pu
      | %<angleLF>deg.
      | %<Name>
  bus83 : powerlib/Measurements/Load Flow Bus  LConnTagsString=a  Phases=single  Connectors=on one side  ID=bus83  Vbase=225000  Vref=1  Vangle=0  VLF=1  VLFb=1  VLFc=1  angleLF=0  angleLFb=0  angleLFc=0
      settings: AttributesFormatString=|
      | %<ID>
      | %<Vbase>V
      | %<VLF>pu
      | %<angleLF>deg.
      | %<Name>
  bus84 : powerlib/Measurements/Load Flow Bus  LConnTagsString=a  Phases=single  Connectors=on one side  ID=bus84  Vbase=225000  Vref=1  Vangle=0  VLF=1  VLFb=1  VLFc=1  angleLF=0  angleLFb=0  angleLFc=0
      settings: AttributesFormatString=|
      | %<ID>
      | %<Vbase>V
      | %<VLF>pu
      | %<angleLF>deg.
      | %<Name>
  bus85 : powerlib/Measurements/Load Flow Bus  LConnTagsString=a  Phases=single  Connectors=on one side  ID=bus85  Vbase=225000  Vref=1  Vangle=0  VLF=1  VLFb=1  VLFc=1  angleLF=0  angleLFb=0  angleLFc=0
      settings: AttributesFormatString=|
      | %<ID>
      | %<Vbase>V
      | %<VLF>pu
      | %<angleLF>deg.
      | %<Name>
  bus9 : powerlib/Measurements/Load Flow Bus  LConnTagsString=a  Phases=single  Connectors=on one side  ID=bus9  Vbase=150000  Vref=1  Vangle=0  VLF=1  VLFb=1  VLFc=1  angleLF=0  angleLFb=0  angleLFc=0
      settings: AttributesFormatString=|
      | %<ID>
      | %<Vbase>V
      | %<VLF>pu
      | %<angleLF>deg.
      | %<Name>
  ligne_150_Kv_Diviation_Midoun_CN_215133456_150000_CN_198577383_150000 : powerlib/Elements/Distributed Parameters Line  Phases=3  Frequency=50  Resistance=[0.01273 0.3864]  Inductance="[0.9337e-3  4.1264e-3]"  Capacitance=[12.74e-9 7.751e-9]  Length=24.3241  x1=[8.73114913702011e-11 380000 380000;314.159265358979 314.159265358979 314.159265358979;-0.177670123217348 0.415246442777429 -1.15554988401747]  x2=[1.26090477118469e-09 381852.398472139 381852.398472139;314.159265358979 314.159265358979 314.159265358979;-1.41941675517191 0.415007521738739 -1.15578880505616]  x3=[1.07663708898761e-11 1405.24743813465 1405.24743813466;314.159265358979 314.159265358979 314.159265358979;-2.70558821102223 0.316110507002444 -1.25468581979246]  x4=[8.62234243168895e-12 1405.96374414071 1405.9637441407;314.159265358979 314.159265358979 314.159265358979;0.245769282942371 0.405640215255436 -1.16515611153945]  x5=0.000565541566995742  V1=ones(3,3)  V2=ones(3,3)  I1=ones(3,3)  I2=ones(3,3)  nHarmo=1  Measurements=None
  ligne_150_Kv_Diviation_Midoun_CN_215133456_150000_CN_242384114_150000 : powerlib/Elements/Distributed Parameters Line  Phases=3  Frequency=50  Resistance=[0.01273 0.3864]  Inductance="[0.9337e-3  4.1264e-3]"  Capacitance=[12.74e-9 7.751e-9]  Length=41.6444  x1=[8.73114913702011e-11 380000 380000;314.159265358979 314.159265358979 314.159265358979;-0.177670123217348 0.415246442777429 -1.15554988401747]  x2=[1.26090477118469e-09 381852.398472139 381852.398472139;314.159265358979 314.159265358979 314.159265358979;-1.41941675517191 0.415007521738739 -1.15578880505616]  x3=[1.07663708898761e-11 1405.24743813465 1405.24743813466;314.159265358979 314.159265358979 314.159265358979;-2.70558821102223 0.316110507002444 -1.25468581979246]  x4=[8.62234243168895e-12 1405.96374414071 1405.9637441407;314.159265358979 314.159265358979 314.159265358979;0.245769282942371 0.405640215255436 -1.16515611153945]  x5=0.000565541566995742  V1=ones(3,3)  V2=ones(3,3)  I1=ones(3,3)  I2=ones(3,3)  nHarmo=1  Measurements=None
  ligne_150_Kv_Ghannouch_Robbana_CN_242390602_150000_CN_198577383_150000 : powerlib/Elements/Distributed Parameters Line  Phases=3  Frequency=50  Resistance=[0.01273 0.3864]  Inductance="[0.9337e-3  4.1264e-3]"  Capacitance=[12.74e-9 7.751e-9]  Length=18.8387  x1=[8.73114913702011e-11 380000 380000;314.159265358979 314.159265358979 314.159265358979;-0.177670123217348 0.415246442777429 -1.15554988401747]  x2=[1.26090477118469e-09 381852.398472139 381852.398472139;314.159265358979 314.159265358979 314.159265358979;-1.41941675517191 0.415007521738739 -1.15578880505616]  x3=[1.07663708898761e-11 1405.24743813465 1405.24743813466;314.159265358979 314.159265358979 314.159265358979;-2.70558821102223 0.316110507002444 -1.25468581979246]  x4=[8.62234243168895e-12 1405.96374414071 1405.9637441407;314.159265358979 314.159265358979 314.159265358979;0.245769282942371 0.405640215255436 -1.16515611153945]  x5=0.000565541566995742  V1=ones(3,3)  V2=ones(3,3)  I1=ones(3,3)  I2=ones(3,3)  nHarmo=1  Measurements=None
  powergui : powerlib/powergui  Priority=1  SimulationMode=Phasor  SolverType=Tustin/Backward Euler (TBE)  SampleTime=50e-6  frequency=50  SPID=off  DisableSnubberDevices=off  DisableRonSwitches=off  DisableVfSwitches=off  SwTol=0  DisplayEquations=off  Interpol=off  ExternalGateDelay=off  methode=off  Ts=10  FunctionMessages=off  echomessages=off  HookPort=off  EnableUseOfTLC=off  x0status=blocks  frequencyindice=50  Pbase=3000e6  ErrMax=0.0001  Iterations=50  UnitsV=V  UnitsW=W  buscounter=0  RestoreLinks=warning  ResistiveCurrentMeasurement=off  Frange=[0:2:500]  Ylog=off  Xlog=on  ShowGrid=off  save=off  variable=ZData  structure=0  ZoomFFT=off  StartTime=0.0  cycles=1  DisplayStyle=1  fundamental=60  FreqAxis=off  MaxFrequency=1000  frequencyindicesteady=1  RmsSteady=1  display=off
  connections:
  LIGNE_150_Kv_MSAKEN_NORD_MSAKEN_3_CN_28943745_150000_CN_130775787_150000/LConn1 -- T_28943745__POSTE_MSAKEN_NORD/RConn1 -- LIGNE_150_Kv_SOUSSE_MSAKEN_NORD_CN_28943745_150000_CN_111375430_150000/LConn1 -- L_28943745/LConn1
  LIGNE_150_Kv_MSAKEN_NORD_MSAKEN_3_CN_28943745_150000_CN_130775787_150000/LConn2 -- T_28943745__POSTE_MSAKEN_NORD/RConn2 -- LIGNE_150_Kv_SOUSSE_MSAKEN_NORD_CN_28943745_150000_CN_111375430_150000/LConn2 -- L_28943745/LConn2
  LIGNE_150_Kv_MSAKEN_NORD_MSAKEN_3_CN_28943745_150000_CN_130775787_150000/LConn3 -- T_28943745__POSTE_MSAKEN_NORD/RConn3 -- LIGNE_150_Kv_SOUSSE_MSAKEN_NORD_CN_28943745_150000_CN_111375430_150000/LConn3 -- L_28943745/LConn3 -- bus1/LConn1
  LIGNE_150_Kv_MSAKEN_NORD_MSAKEN_3_CN_28943745_150000_CN_130775787_150000/RConn1 -- T_130775787__POSTE_MSAKEN/LConn1 -- LIGNE_150_Kv__MSAKEN_ELJEM_CN_178549814_150000_CN_130775787_150000/LConn1
  LIGNE_150_Kv_MSAKEN_NORD_MSAKEN_3_CN_28943745_150000_CN_130775787_150000/RConn2 -- T_130775787__POSTE_MSAKEN/LConn2 -- LIGNE_150_Kv__MSAKEN_ELJEM_CN_178549814_150000_CN_130775787_150000/LConn2
  LIGNE_150_Kv_MSAKEN_NORD_MSAKEN_3_CN_28943745_150000_CN_130775787_150000/RConn3 -- T_130775787__POSTE_MSAKEN/LConn3 -- LIGNE_150_Kv__MSAKEN_ELJEM_CN_178549814_150000_CN_130775787_150000/LConn3 -- bus2/LConn1
  LIGNE_150_Kv_SOUSSE_MSAKEN_NORD_CN_28943745_150000_CN_111375430_150000/RConn1 -- T_111375430__/LConn1 -- LIGNE_225_Kv_SOUSSE__MOKNINE_CN_111375430_150000_CN_178326515_150000/LConn1
  LIGNE_150_Kv_SOUSSE_MSAKEN_NORD_CN_28943745_150000_CN_111375430_150000/RConn2 -- T_111375430__/LConn2 -- LIGNE_225_Kv_SOUSSE__MOKNINE_CN_111375430_150000_CN_178326515_150000/LConn2
  LIGNE_150_Kv_SOUSSE_MSAKEN_NORD_CN_28943745_150000_CN_111375430_150000/RConn3 -- T_111375430__/LConn3 -- LIGNE_225_Kv_SOUSSE__MOKNINE_CN_111375430_150000_CN_178326515_150000/LConn3 -- bus3/LConn1
  LIGNE_150_Kv_SFAX_SIDI_MANSOUR_CN_178543491_150000_CN_178549814_150000/LConn1 -- T_178543491__POSTE_GREMDA/LConn1 -- LIGNE_150_Kv_SFAX_THYNA_CN_178543491_150000_CN_201812735_150000/LConn1 -- LIGNE_150_Kv_SFAX_THYNA_CN_178543491_150000_CN_178547287_150000/LConn1
  LIGNE_150_Kv_SFAX_SIDI_MANSOUR_CN_178543491_150000_CN_178549814_150000/LConn2 -- T_178543491__POSTE_GREMDA/LConn2 -- LIGNE_150_Kv_SFAX_THYNA_CN_178543491_150000_CN_201812735_150000/LConn2 -- LIGNE_150_Kv_SFAX_THYNA_CN_178543491_150000_CN_178547287_150000/LConn2
  LIGNE_150_Kv_SFAX_SIDI_MANSOUR_CN_178543491_150000_CN_178549814_150000/LConn3 -- T_178543491__POSTE_GREMDA/LConn3 -- LIGNE_150_Kv_SFAX_THYNA_CN_178543491_150000_CN_201812735_150000/LConn3 -- LIGNE_150_Kv_SFAX_THYNA_CN_178543491_150000_CN_178547287_150000/LConn3 -- bus4/LConn1
  LIGNE_150_Kv_SFAX_SIDI_MANSOUR_CN_178543491_150000_CN_178549814_150000/RConn1 -- T_178549814__POSTE_ELJEM/LConn1 -- LIGNE_150_Kv_MOKNINE_ELJEM_CN_178549814_150000_CN_178326515_150000/LConn1 -- LIGNE_150_Kv__MSAKEN_ELJEM_CN_178549814_150000_CN_130775787_150000/RConn1
  LIGNE_150_Kv_SFAX_SIDI_MANSOUR_CN_178543491_150000_CN_178549814_150000/RConn2 -- T_178549814__POSTE_ELJEM/LConn2 -- LIGNE_150_Kv_MOKNINE_ELJEM_CN_178549814_150000_CN_178326515_150000/LConn2 -- LIGNE_150_Kv__MSAKEN_ELJEM_CN_178549814_150000_CN_130775787_150000/RConn2
  LIGNE_150_Kv_SFAX_SIDI_MANSOUR_CN_178543491_150000_CN_178549814_150000/RConn3 -- T_178549814__POSTE_ELJEM/LConn3 -- LIGNE_150_Kv_MOKNINE_ELJEM_CN_178549814_150000_CN_178326515_150000/LConn3 -- bus5/LConn1 -- LIGNE_150_Kv__MSAKEN_ELJEM_CN_178549814_150000_CN_130775787_150000/RConn3
  LIGNE_150_Kv_SFAX_THYNA_CN_178543491_150000_CN_201812735_150000/RConn1 -- T_201812735__POSTE_MEKNASSY/RConn1 -- LIGNE_150_Kv_DIV_SKHIRA_CN_202286224_150000_CN_201812735_150000/LConn1 -- LIGNE_150_Kv_MEKNASSY_SIDI_BOUZID_CN_174150822_150000_CN_201812735_150000/LConn1 -- L_201812735/LConn1
  LIGNE_150_Kv_SFAX_THYNA_CN_178543491_150000_CN_201812735_150000/RConn2 -- T_201812735__POSTE_MEKNASSY/RConn2 -- LIGNE_150_Kv_DIV_SKHIRA_CN_202286224_150000_CN_201812735_150000/LConn2 -- LIGNE_150_Kv_MEKNASSY_SIDI_BOUZID_CN_174150822_150000_CN_201812735_150000/LConn2 -- L_201812735/LConn2
  LIGNE_150_Kv_SFAX_THYNA_CN_178543491_150000_CN_201812735_150000/RConn3 -- T_201812735__POSTE_MEKNASSY/RConn3 -- LIGNE_150_Kv_DIV_SKHIRA_CN_202286224_150000_CN_201812735_150000/LConn3 -- LIGNE_150_Kv_MEKNASSY_SIDI_BOUZID_CN_174150822_150000_CN_201812735_150000/LConn3 -- L_201812735/LConn3 -- bus6/LConn1
  T_178547287__POSTE_THYNA/LConn1 -- LIGNE_150_Kv_SFAX_THYNA_CN_178543491_150000_CN_178547287_150000/RConn1
  T_178547287__POSTE_THYNA/LConn2 -- LIGNE_150_Kv_SFAX_THYNA_CN_178543491_150000_CN_178547287_150000/RConn2
  LIGNE_150_Kv_SFAX_THYNA_CN_178543491_150000_CN_178547287_150000/RConn3 -- T_178547287__POSTE_THYNA/LConn3 -- bus7/LConn1
  T_322419513__POSTE_DE_LA_CIMENTERIE_DE_GABES/LConn1 -- LIGNE_150_Kv_BOUCHEMMA_CIMENTERIE_DE_GABES_CN_322419513_150000_CN_189193656_150000/LConn1
  T_322419513__POSTE_DE_LA_CIMENTERIE_DE_GABES/LConn2 -- LIGNE_150_Kv_BOUCHEMMA_CIMENTERIE_DE_GABES_CN_322419513_150000_CN_189193656_150000/LConn2
  LIGNE_150_Kv_BOUCHEMMA_CIMENTERIE_DE_GABES_CN_322419513_150000_CN_189193656_150000/LConn3 -- T_322419513__POSTE_DE_LA_CIMENTERIE_DE_GABES/LConn3 -- bus8/LConn1
  LIGNE_150_Kv_BOUCHEMMA_CIMENTERIE_DE_GABES_CN_322419513_150000_CN_189193656_150000/RConn1 -- T_189193656__/RConn1 -- LIGNE_150_Kv_BOUCHEMMA_KEBILI_CN_189193656_150000_CN_253586233_150000/LConn1 -- L_189193656/LConn1 -- _CN_189193656_150000_CN_242390602_150000/LConn1 -- LIGNE_150_Kv_BOUCHEMMA_GABES_SUD_CN_189193656_150000_CN_242392536_150000/LConn1 -- LIGNE_150_Kv_DIV_SKHIRA_CN_202286224_150000_CN_189193656_150000/LConn1 -- _CN_189193656_150000_CN_206449367_150000/LConn1
  LIGNE_150_Kv_BOUCHEMMA_CIMENTERIE_DE_GABES_CN_322419513_150000_CN_189193656_150000/RConn2 -- T_189193656__/RConn2 -- LIGNE_150_Kv_BOUCHEMMA_KEBILI_CN_189193656_150000_CN_253586233_150000/LConn2 -- L_189193656/LConn2 -- _CN_189193656_150000_CN_242390602_150000/LConn2 -- LIGNE_150_Kv_BOUCHEMMA_GABES_SUD_CN_189193656_150000_CN_242392536_150000/LConn2 -- LIGNE_150_Kv_DIV_SKHIRA_CN_202286224_150000_CN_189193656_150000/LConn2 -- _CN_189193656_150000_CN_206449367_150000/LConn2
  LIGNE_150_Kv_BOUCHEMMA_CIMENTERIE_DE_GABES_CN_322419513_150000_CN_189193656_150000/RConn3 -- T_189193656__/RConn3 -- LIGNE_150_Kv_BOUCHEMMA_KEBILI_CN_189193656_150000_CN_253586233_150000/LConn3 -- L_189193656/LConn3 -- bus9/LConn1 -- _CN_189193656_150000_CN_242390602_150000/LConn3 -- LIGNE_150_Kv_BOUCHEMMA_GABES_SUD_CN_189193656_150000_CN_242392536_150000/LConn3 -- LIGNE_150_Kv_DIV_SKHIRA_CN_202286224_150000_CN_189193656_150000/LConn3 -- _CN_189193656_150000_CN_206449367_150000/LConn3
  LIGNE_150_Kv_DIV_SKHIRA_CN_202286224_150000_CN_201812735_150000/RConn1 -- T_202286224__POSTE_SKHIRA/LConn1 -- LIGNE_150_Kv_DIV_SKHIRA_CN_202286224_150000_CN_189193656_150000/RConn1 -- LIGNE_150_Kv_DIV_SKHIRA_CN_202286224_150000_CN_242390602_150000/LConn1
  LIGNE_150_Kv_DIV_SKHIRA_CN_202286224_150000_CN_201812735_150000/RConn2 -- T_202286224__POSTE_SKHIRA/LConn2 -- LIGNE_150_Kv_DIV_SKHIRA_CN_202286224_150000_CN_189193656_150000/RConn2 -- LIGNE_150_Kv_DIV_SKHIRA_CN_202286224_150000_CN_242390602_150000/LConn2
  LIGNE_150_Kv_DIV_SKHIRA_CN_202286224_150000_CN_201812735_150000/RConn3 -- T_202286224__POSTE_SKHIRA/LConn3 -- LIGNE_150_Kv_DIV_SKHIRA_CN_202286224_150000_CN_189193656_150000/RConn3 -- LIGNE_150_Kv_DIV_SKHIRA_CN_202286224_150000_CN_242390602_150000/LConn3 -- bus10/LConn1
  LIGNE_150_Kv_DIV_SKHIRA_CN_202286224_150000_CN_242390602_150000/RConn1 -- T_242390602__POSTE_DE_GHANNOUCH/LConn1 -- ligne_150_Kv_Ghannouch_Robbana_CN_242390602_150000_CN_198577383_150000/LConn1 -- _CN_189193656_150000_CN_242390602_150000/RConn1
  LIGNE_150_Kv_DIV_SKHIRA_CN_202286224_150000_CN_242390602_150000/RConn2 -- T_242390602__POSTE_DE_GHANNOUCH/LConn2 -- ligne_150_Kv_Ghannouch_Robbana_CN_242390602_150000_CN_198577383_150000/LConn2 -- _CN_189193656_150000_CN_242390602_150000/RConn2
  LIGNE_150_Kv_DIV_SKHIRA_CN_202286224_150000_CN_242390602_150000/RConn3 -- T_242390602__POSTE_DE_GHANNOUCH/LConn3 -- ligne_150_Kv_Ghannouch_Robbana_CN_242390602_150000_CN_198577383_150000/LConn3 -- bus11/LConn1 -- _CN_189193656_150000_CN_242390602_150000/RConn3
  Ligne_150_KV_Feriana_Mdhilla_CN_252371715_150000_CN_206449367_150000/LConn1 -- T_252371715__POSTE_FERIANA/LConn1 -- _CN_252371715_150000_CN_206389818_150000/LConn1
  Ligne_150_KV_Feriana_Mdhilla_CN_252371715_150000_CN_206449367_150000/LConn2 -- T_252371715__POSTE_FERIANA/LConn2 -- _CN_252371715_150000_CN_206389818_150000/LConn2
  Ligne_150_KV_Feriana_Mdhilla_CN_252371715_150000_CN_206449367_150000/LConn3 -- T_252371715__POSTE_FERIANA/LConn3 -- _CN_252371715_150000_CN_206389818_150000/LConn3 -- bus12/LConn1
  Ligne_150_KV_Feriana_Mdhilla_CN_252371715_150000_CN_206449367_150000/RConn1 -- T_206449367_150000_POSTE_DE_MDHILLA/LConn1 -- LIGNE_150_KV_METLAOUI_DIV_MDHILLA_CN_206389818_150000_CN_206449367_150000/LConn1 -- _CN_189193656_150000_CN_206449367_150000/RConn1
  Ligne_150_KV_Feriana_Mdhilla_CN_252371715_150000_CN_206449367_150000/RConn2 -- T_206449367_150000_POSTE_DE_MDHILLA/LConn2 -- LIGNE_150_KV_METLAOUI_DIV_MDHILLA_CN_206389818_150000_CN_206449367_150000/LConn2 -- _CN_189193656_150000_CN_206449367_150000/RConn2
  Ligne_150_KV_Feriana_Mdhilla_CN_252371715_150000_CN_206449367_150000/RConn3 -- T_206449367_150000_POSTE_DE_MDHILLA/LConn3 -- LIGNE_150_KV_METLAOUI_DIV_MDHILLA_CN_206389818_150000_CN_206449367_150000/LConn3 -- bus13/LConn1 -- _CN_189193656_150000_CN_206449367_150000/RConn3
  _CN_252371715_150000_CN_206389818_150000/RConn1 -- T_206389818__POSTE_METLAOUI/LConn1 -- LIGNE_150_KV_METLAOUI_DIV_MDHILLA_CN_206389818_150000_CN_206449367_150000/RConn1 -- LIGNE_150_KV_METLAOUI_TOZEUR_CN_207339172_150000_CN_206389818_150000/LConn1
  _CN_252371715_150000_CN_206389818_150000/RConn2 -- T_206389818__POSTE_METLAOUI/LConn2 -- LIGNE_150_KV_METLAOUI_DIV_MDHILLA_CN_206389818_150000_CN_206449367_150000/RConn2 -- LIGNE_150_KV_METLAOUI_TOZEUR_CN_207339172_150000_CN_206389818_150000/LConn2
  _CN_252371715_150000_CN_206389818_150000/RConn3 -- T_206389818__POSTE_METLAOUI/LConn3 -- LIGNE_150_KV_METLAOUI_DIV_MDHILLA_CN_206389818_150000_CN_206449367_150000/RConn3 -- bus14/LConn1 -- LIGNE_150_KV_METLAOUI_TOZEUR_CN_207339172_150000_CN_206389818_150000/LConn3
  T_207339172__POSTE_TOZEUR/LConn1 -- LIGNE_150_KV_METLAOUI_TOZEUR_CN_207339172_150000_CN_206389818_150000/RConn1
  T_207339172__POSTE_TOZEUR/LConn2 -- LIGNE_150_KV_METLAOUI_TOZEUR_CN_207339172_150000_CN_206389818_150000/RConn2
  LIGNE_150_KV_METLAOUI_TOZEUR_CN_207339172_150000_CN_206389818_150000/RConn3 -- T_207339172__POSTE_TOZEUR/LConn3 -- bus15/LConn1
  T_174150822__POSTE_LESSOUDA/LConn1 -- LIGNE_150_Kv_MEKNASSY_SIDI_BOUZID_CN_174150822_150000_CN_201812735_150000/RConn1
  T_174150822__POSTE_LESSOUDA/LConn2 -- LIGNE_150_Kv_MEKNASSY_SIDI_BOUZID_CN_174150822_150000_CN_201812735_150000/RConn2
  LIGNE_150_Kv_MEKNASSY_SIDI_BOUZID_CN_174150822_150000_CN_201812735_150000/RConn3 -- T_174150822__POSTE_LESSOUDA/LConn3 -- bus16/LConn1
  T_131220525__Poste__Enfidha_Sud/LConn1 -- LIGNE_150_Kv_ENFIDHA_DIV_BOUFICHA_CN_131220525_150000_CN_106469430_150000/LConn1
  T_131220525__Poste__Enfidha_Sud/LConn2 -- LIGNE_150_Kv_ENFIDHA_DIV_BOUFICHA_CN_131220525_150000_CN_106469430_150000/LConn2
  LIGNE_150_Kv_ENFIDHA_DIV_BOUFICHA_CN_131220525_150000_CN_106469430_150000/LConn3 -- T_131220525__Poste__Enfidha_Sud/LConn3 -- bus17/LConn1
  LIGNE_150_Kv_ENFIDHA_DIV_BOUFICHA_CN_131220525_150000_CN_106469430_150000/RConn1 -- T_106469430__POSTE_BOUFICHA/RConn1 -- L_106469430/LConn1
  LIGNE_150_Kv_ENFIDHA_DIV_BOUFICHA_CN_131220525_150000_CN_106469430_150000/RConn2 -- T_106469430__POSTE_BOUFICHA/RConn2 -- L_106469430/LConn2
  LIGNE_150_Kv_ENFIDHA_DIV_BOUFICHA_CN_131220525_150000_CN_106469430_150000/RConn3 -- T_106469430__POSTE_BOUFICHA/RConn3 -- L_106469430/LConn3 -- bus18/LConn1
  T_242392536__POSTE_GABES_SUD/LConn1 -- LIGNE_150_Kv_BOUCHEMMA_GABES_SUD_CN_189193656_150000_CN_242392536_150000/RConn1
  T_242392536__POSTE_GABES_SUD/LConn2 -- LIGNE_150_Kv_BOUCHEMMA_GABES_SUD_CN_189193656_150000_CN_242392536_150000/RConn2
  LIGNE_150_Kv_BOUCHEMMA_GABES_SUD_CN_189193656_150000_CN_242392536_150000/RConn3 -- T_242392536__POSTE_GABES_SUD/LConn3 -- bus19/LConn1
  T_253586233__POSTE_DE_KEBILI/LConn1 -- LIGNE_150_Kv_BOUCHEMMA_KEBILI_CN_189193656_150000_CN_253586233_150000/RConn1
  T_253586233__POSTE_DE_KEBILI/LConn2 -- LIGNE_150_Kv_BOUCHEMMA_KEBILI_CN_189193656_150000_CN_253586233_150000/RConn2
  LIGNE_150_Kv_BOUCHEMMA_KEBILI_CN_189193656_150000_CN_253586233_150000/RConn3 -- T_253586233__POSTE_DE_KEBILI/LConn3 -- bus20/LConn1
  LIGNE_150_Kv_MOKNINE_ELJEM_CN_178549814_150000_CN_178326515_150000/RConn1 -- T_178326515__POSTE_MOKNINE/RConn1 -- LIGNE_225_Kv_SOUSSE__MOKNINE_CN_111375430_150000_CN_178326515_150000/RConn1 -- L_178326515/LConn1
  LIGNE_150_Kv_MOKNINE_ELJEM_CN_178549814_150000_CN_178326515_150000/RConn2 -- T_178326515__POSTE_MOKNINE/RConn2 -- LIGNE_225_Kv_SOUSSE__MOKNINE_CN_111375430_150000_CN_178326515_150000/RConn2 -- L_178326515/LConn2
  LIGNE_150_Kv_MOKNINE_ELJEM_CN_178549814_150000_CN_178326515_150000/RConn3 -- T_178326515__POSTE_MOKNINE/RConn3 -- LIGNE_225_Kv_SOUSSE__MOKNINE_CN_111375430_150000_CN_178326515_150000/RConn3 -- L_178326515/LConn3 -- bus21/LConn1
  ligne_150_Kv_Ghannouch_Robbana_CN_242390602_150000_CN_198577383_150000/RConn1 -- T_198577383__POSTE_ROBBANA/LConn1 -- ligne_150_Kv_Diviation_Midoun_CN_215133456_150000_CN_198577383_150000/LConn1
  ligne_150_Kv_Ghannouch_Robbana_CN_242390602_150000_CN_198577383_150000/RConn2 -- T_198577383__POSTE_ROBBANA/LConn2 -- ligne_150_Kv_Diviation_Midoun_CN_215133456_150000_CN_198577383_150000/LConn2
  ligne_150_Kv_Ghannouch_Robbana_CN_242390602_150000_CN_198577383_150000/RConn3 -- T_198577383__POSTE_ROBBANA/LConn3 -- ligne_150_Kv_Diviation_Midoun_CN_215133456_150000_CN_198577383_150000/LConn3 -- bus22/LConn1
  ligne_150_Kv_Diviation_Midoun_CN_215133456_150000_CN_242384114_150000/LConn1 -- T_215133456__POSTE_MIDOUN/LConn1 -- ligne_150_Kv_Diviation_Midoun_CN_215133456_150000_CN_198577383_150000/RConn1
  ligne_150_Kv_Diviation_Midoun_CN_215133456_150000_CN_242384114_150000/LConn2 -- T_215133456__POSTE_MIDOUN/LConn2 -- ligne_150_Kv_Diviation_Midoun_CN_215133456_150000_CN_198577383_150000/RConn2
  ligne_150_Kv_Diviation_Midoun_CN_215133456_150000_CN_242384114_150000/LConn3 -- T_215133456__POSTE_MIDOUN/LConn3 -- ligne_150_Kv_Diviation_Midoun_CN_215133456_150000_CN_198577383_150000/RConn3 -- bus23/LConn1
  T_242384114__POSTE_ZARZIS/LConn1 -- ligne_150_Kv_Diviation_Midoun_CN_215133456_150000_CN_242384114_150000/RConn1
  T_242384114__POSTE_ZARZIS/LConn2 -- ligne_150_Kv_Diviation_Midoun_CN_215133456_150000_CN_242384114_150000/RConn2
  ligne_150_Kv_Diviation_Midoun_CN_215133456_150000_CN_242384114_150000/RConn3 -- T_242384114__POSTE_ZARZIS/LConn3 -- bus24/LConn1
  LIGNE_225_Kv_SIDI_MANSOUR_MSAKEN_NORD_CN_28943745_225000_CN_178328237_225000/LConn1 -- T_28943745__POSTE_MSAKEN_NORD/LConn1 -- _CN_28943745_225000_CN_224416644_225000/LConn1 -- _CN_28943745_225000_CN_111375420_225000/LConn1
  LIGNE_225_Kv_SIDI_MANSOUR_MSAKEN_NORD_CN_28943745_225000_CN_178328237_225000/LConn2 -- T_28943745__POSTE_MSAKEN_NORD/LConn2 -- _CN_28943745_225000_CN_224416644_225000/LConn2 -- _CN_28943745_225000_CN_111375420_225000/LConn2
  LIGNE_225_Kv_SIDI_MANSOUR_MSAKEN_NORD_CN_28943745_225000_CN_178328237_225000/LConn3 -- T_28943745__POSTE_MSAKEN_NORD/LConn3 -- _CN_28943745_225000_CN_224416644_225000/LConn3 -- bus25/LConn1 -- _CN_28943745_225000_CN_111375420_225000/LConn3
  LIGNE_225_Kv_SIDI_MANSOUR_MSAKEN_NORD_CN_28943745_225000_CN_178328237_225000/RConn1 -- T_178328237__POSTE_SIDI_MANSOUR/LConn1 -- LIGNE_225_Kv_SIDI_MANSOUR_DIV_MOKNINE_CN_178328237_225000_CN_178326515_225000/LConn1 -- LIGNE_225_Kv_SIDI_MANSOUR_DIV_MOKNINE_CN_178328237_225000_CN_111375420_225000/LConn1 -- _CN_178328237_225000_CN_189193646_225000/LConn1
  LIGNE_225_Kv_SIDI_MANSOUR_MSAKEN_NORD_CN_28943745_225000_CN_178328237_225000/RConn2 -- T_178328237__POSTE_SIDI_MANSOUR/LConn2 -- LIGNE_225_Kv_SIDI_MANSOUR_DIV_MOKNINE_CN_178328237_225000_CN_178326515_225000/LConn2 -- LIGNE_225_Kv_SIDI_MANSOUR_DIV_MOKNINE_CN_178328237_225000_CN_111375420_225000/LConn2 -- _CN_178328237_225000_CN_189193646_225000/LConn2
  LIGNE_225_Kv_SIDI_MANSOUR_MSAKEN_NORD_CN_28943745_225000_CN_178328237_225000/RConn3 -- T_178328237__POSTE_SIDI_MANSOUR/LConn3 -- LIGNE_225_Kv_SIDI_MANSOUR_DIV_MOKNINE_CN_178328237_225000_CN_178326515_225000/LConn3 -- LIGNE_225_Kv_SIDI_MANSOUR_DIV_MOKNINE_CN_178328237_225000_CN_111375420_225000/LConn3 -- _CN_178328237_225000_CN_189193646_225000/LConn3 -- bus26/LConn1
  _CN_28943745_225000_CN_111375420_225000/RConn1 -- T_111375420__POSTE_SOUSSE/LConn1 -- LIGNE_225_Kv_SIDI_MANSOUR_DIV_MOKNINE_CN_178328237_225000_CN_111375420_225000/RConn1 -- LIGNE_225_Kv_SOUSSE_NAASAN_CN_111375420_225000_CN_125504235_225000/LConn1
  _CN_28943745_225000_CN_111375420_225000/RConn2 -- T_111375420__POSTE_SOUSSE/LConn2 -- LIGNE_225_Kv_SIDI_MANSOUR_DIV_MOKNINE_CN_178328237_225000_CN_111375420_225000/RConn2 -- LIGNE_225_Kv_SOUSSE_NAASAN_CN_111375420_225000_CN_125504235_225000/LConn2
  _CN_28943745_225000_CN_111375420_225000/RConn3 -- T_111375420__POSTE_SOUSSE/LConn3 -- LIGNE_225_Kv_SIDI_MANSOUR_DIV_MOKNINE_CN_178328237_225000_CN_111375420_225000/RConn3 -- LIGNE_225_Kv_SOUSSE_NAASAN_CN_111375420_225000_CN_125504235_225000/LConn3 -- bus27/LConn1
  _CN_28943745_225000_CN_224416644_225000/RConn1 -- T_224416644__POSTE_OUESLATIA/LConn1 -- LIGNE_225_Kv_OUESLATIA_HAJEB_LAYOUN_CN_224416644_225000_CN_224417135_225000/LConn1 -- LIGNE_225_Kv_OUESLATIA_BIR_MCHARGA_CN_224416644_225000_CN_173531194_225000/LConn1
  _CN_28943745_225000_CN_224416644_225000/RConn2 -- T_224416644__POSTE_OUESLATIA/LConn2 -- LIGNE_225_Kv_OUESLATIA_HAJEB_LAYOUN_CN_224416644_225000_CN_224417135_225000/LConn2 -- LIGNE_225_Kv_OUESLATIA_BIR_MCHARGA_CN_224416644_225000_CN_173531194_225000/LConn2
  _CN_28943745_225000_CN_224416644_225000/RConn3 -- T_224416644__POSTE_OUESLATIA/LConn3 -- LIGNE_225_Kv_OUESLATIA_HAJEB_LAYOUN_CN_224416644_225000_CN_224417135_225000/LConn3 -- LIGNE_225_Kv_OUESLATIA_BIR_MCHARGA_CN_224416644_225000_CN_173531194_225000/LConn3 -- bus28/LConn1
  LIGNE_225_Kv_OUESLATIA_HAJEB_LAYOUN_CN_224416644_225000_CN_224417135_225000/RConn1 -- T_224417135__POSTE_HAJEB_LAYOUN/LConn1 -- LIGNE_150_Kv_MEKNASSY_HAJEB_LAYOUN_CN_224417135_225000_CN_201812735_225000/LConn1
  LIGNE_225_Kv_OUESLATIA_HAJEB_LAYOUN_CN_224416644_225000_CN_224417135_225000/RConn2 -- T_224417135__POSTE_HAJEB_LAYOUN/LConn2 -- LIGNE_150_Kv_MEKNASSY_HAJEB_LAYOUN_CN_224417135_225000_CN_201812735_225000/LConn2
  LIGNE_225_Kv_OUESLATIA_HAJEB_LAYOUN_CN_224416644_225000_CN_224417135_225000/RConn3 -- T_224417135__POSTE_HAJEB_LAYOUN/LConn3 -- LIGNE_150_Kv_MEKNASSY_HAJEB_LAYOUN_CN_224417135_225000_CN_201812735_225000/LConn3 -- bus29/LConn1
  LIGNE_225_Kv_OUESLATIA_BIR_MCHARGA_CN_224416644_225000_CN_173531194_225000/RConn1 -- T_173531194__POSTE_BIR_MCHARGA/LConn1 -- LIGNE_225_Kv__BOUFICHA_ZAGHOUAN_CN_106469430_225000_CN_173531194_225000/LConn1 -- LIGNE_225_Kv_NAASAN_BIR_MCHARGA_CN_173531194_225000_CN_125504235_225000/LConn1 -- _CN_129996167_225000_CN_173531194_225000/LConn1
  LIGNE_225_Kv_OUESLATIA_BIR_MCHARGA_CN_224416644_225000_CN_173531194_225000/RConn2 -- T_173531194__POSTE_BIR_MCHARGA/LConn2 -- LIGNE_225_Kv__BOUFICHA_ZAGHOUAN_CN_106469430_225000_CN_173531194_225000/LConn2 -- LIGNE_225_Kv_NAASAN_BIR_MCHARGA_CN_173531194_225000_CN_125504235_225000/LConn2 -- _CN_129996167_225000_CN_173531194_225000/LConn2
  LIGNE_225_Kv_OUESLATIA_BIR_MCHARGA_CN_224416644_225000_CN_173531194_225000/RConn3 -- T_173531194__POSTE_BIR_MCHARGA/LConn3 -- LIGNE_225_Kv__BOUFICHA_ZAGHOUAN_CN_106469430_225000_CN_173531194_225000/LConn3 -- LIGNE_225_Kv_NAASAN_BIR_MCHARGA_CN_173531194_225000_CN_125504235_225000/LConn3 -- bus30/LConn1 -- _CN_129996167_225000_CN_173531194_225000/LConn3
  LIGNE_400_Kv_MATEUR_MORNAGUIA_CN_129996167_225000_CN_129996179_225000/LConn1 -- T_129996167__/LConn1 -- _CN_129996167_225000_CN_101404944_225000/LConn1 -- _CN_129996167_225000_CN_173531194_225000/RConn1 -- DIV_225_Kv_MORNAGUIA_(_MNIHLA_1_BIR_MCHARGA)_CN_129996167_225000_CN_125504235_225000/LConn1
  LIGNE_400_Kv_MATEUR_MORNAGUIA_CN_129996167_225000_CN_129996179_225000/LConn2 -- T_129996167__/LConn2 -- _CN_129996167_225000_CN_101404944_225000/LConn2 -- _CN_129996167_225000_CN_173531194_225000/RConn2 -- DIV_225_Kv_MORNAGUIA_(_MNIHLA_1_BIR_MCHARGA)_CN_129996167_225000_CN_125504235_225000/LConn2
  LIGNE_400_Kv_MATEUR_MORNAGUIA_CN_129996167_225000_CN_129996179_225000/LConn3 -- T_129996167__/LConn3 -- _CN_129996167_225000_CN_101404944_225000/LConn3 -- _CN_129996167_225000_CN_173531194_225000/RConn3 -- DIV_225_Kv_MORNAGUIA_(_MNIHLA_1_BIR_MCHARGA)_CN_129996167_225000_CN_125504235_225000/LConn3 -- bus31/LConn1
  LIGNE_400_Kv_MATEUR_MORNAGUIA_CN_129996167_225000_CN_129996179_225000/RConn1 -- T_129996179__POSTE_MATEUR/LConn1 -- LIGNE_400_Kv_JANDOUBA_MATEUR_CN_129996179_225000_CN_173534564_225000/LConn1
  LIGNE_400_Kv_MATEUR_MORNAGUIA_CN_129996167_225000_CN_129996179_225000/RConn2 -- T_129996179__POSTE_MATEUR/LConn2 -- LIGNE_400_Kv_JANDOUBA_MATEUR_CN_129996179_225000_CN_173534564_225000/LConn2
  LIGNE_400_Kv_MATEUR_MORNAGUIA_CN_129996167_225000_CN_129996179_225000/RConn3 -- T_129996179__POSTE_MATEUR/LConn3 -- LIGNE_400_Kv_JANDOUBA_MATEUR_CN_129996179_225000_CN_173534564_225000/LConn3 -- bus32/LConn1
  _CN_129996167_225000_CN_101404944_225000/RConn1 -- T_101404944__POSTE_225_90_MNIHLA_1/LConn1 -- _CN_101404944_225000_CN_93164455_225000/LConn1 -- LIGNE_225_Kv_MNIHLA_1_MENZEL_JEMIL_CN_101404944_225000_CN_178494278_225000/LConn1
  _CN_129996167_225000_CN_101404944_225000/RConn2 -- T_101404944__POSTE_225_90_MNIHLA_1/LConn2 -- _CN_101404944_225000_CN_93164455_225000/LConn2 -- LIGNE_225_Kv_MNIHLA_1_MENZEL_JEMIL_CN_101404944_225000_CN_178494278_225000/LConn2
  _CN_129996167_225000_CN_101404944_225000/RConn3 -- T_101404944__POSTE_225_90_MNIHLA_1/LConn3 -- _CN_101404944_225000_CN_93164455_225000/LConn3 -- LIGNE_225_Kv_MNIHLA_1_MENZEL_JEMIL_CN_101404944_225000_CN_178494278_225000/LConn3 -- bus33/LConn1
  DIV_225_Kv_MORNAGUIA_(_MNIHLA_1_BIR_MCHARGA)_CN_129996167_225000_CN_125504235_225000/RConn1 -- T_125504235_225000_POSTE_NAASEN/LConn1 -- LIGNE_225_Kv_RADES_NAASAN_CN_93263381_225000_CN_125504235_225000/LConn1 -- LIGNE_225_Kv_NAASAN_BIR_MCHARGA_CN_173531194_225000_CN_125504235_225000/RConn1 -- LIGNE_225_Kv_SOUSSE_NAASAN_CN_111375420_225000_CN_125504235_225000/RConn1
  DIV_225_Kv_MORNAGUIA_(_MNIHLA_1_BIR_MCHARGA)_CN_129996167_225000_CN_125504235_225000/RConn2 -- T_125504235_225000_POSTE_NAASEN/LConn2 -- LIGNE_225_Kv_RADES_NAASAN_CN_93263381_225000_CN_125504235_225000/LConn2 -- LIGNE_225_Kv_NAASAN_BIR_MCHARGA_CN_173531194_225000_CN_125504235_225000/RConn2 -- LIGNE_225_Kv_SOUSSE_NAASAN_CN_111375420_225000_CN_125504235_225000/RConn2
  DIV_225_Kv_MORNAGUIA_(_MNIHLA_1_BIR_MCHARGA)_CN_129996167_225000_CN_125504235_225000/RConn3 -- T_125504235_225000_POSTE_NAASEN/LConn3 -- LIGNE_225_Kv_RADES_NAASAN_CN_93263381_225000_CN_125504235_225000/LConn3 -- LIGNE_225_Kv_NAASAN_BIR_MCHARGA_CN_173531194_225000_CN_125504235_225000/RConn3 -- LIGNE_225_Kv_SOUSSE_NAASAN_CN_111375420_225000_CN_125504235_225000/RConn3 -- bus34/LConn1
  T_179549833__POSTE_TAJEROUINE_225_KV/LConn1 -- LIGNE_225_Kv_TAJEROUIN_JANDOUBA_CN_179549833_225000_CN_173534564_225000/LConn1
  T_179549833__POSTE_TAJEROUINE_225_KV/LConn2 -- LIGNE_225_Kv_TAJEROUIN_JANDOUBA_CN_179549833_225000_CN_173534564_225000/LConn2
  LIGNE_225_Kv_TAJEROUIN_JANDOUBA_CN_179549833_225000_CN_173534564_225000/LConn3 -- T_179549833__POSTE_TAJEROUINE_225_KV/LConn3 -- bus35/LConn1
  LIGNE_225_Kv_TAJEROUIN_JANDOUBA_CN_179549833_225000_CN_173534564_225000/RConn1 -- T_173534564__POSTE_JENDOUBA/LConn1 -- LIGNE_400_Kv_JANDOUBA_MATEUR_CN_129996179_225000_CN_173534564_225000/RConn1
  LIGNE_225_Kv_TAJEROUIN_JANDOUBA_CN_179549833_225000_CN_173534564_225000/RConn2 -- T_173534564__POSTE_JENDOUBA/LConn2 -- LIGNE_400_Kv_JANDOUBA_MATEUR_CN_129996179_225000_CN_173534564_225000/RConn2
  LIGNE_225_Kv_TAJEROUIN_JANDOUBA_CN_179549833_225000_CN_173534564_225000/RConn3 -- T_173534564__POSTE_JENDOUBA/LConn3 -- LIGNE_400_Kv_JANDOUBA_MATEUR_CN_129996179_225000_CN_173534564_225000/RConn3 -- bus36/LConn1
  G_93164455_/RConn1 -- _CN_101404944_225000_CN_93164455_225000/RConn1
  G_93164455_/RConn2 -- _CN_101404944_225000_CN_93164455_225000/RConn2
  _CN_101404944_225000_CN_93164455_225000/RConn3 -- G_93164455_/RConn3 -- bus37/LConn1
  T_178494278__POSTE_MENZEL_JEMIL/LConn1 -- LIGNE_225_Kv_MNIHLA_1_MENZEL_JEMIL_CN_101404944_225000_CN_178494278_225000/RConn1
  T_178494278__POSTE_MENZEL_JEMIL/LConn2 -- LIGNE_225_Kv_MNIHLA_1_MENZEL_JEMIL_CN_101404944_225000_CN_178494278_225000/RConn2
  LIGNE_225_Kv_MNIHLA_1_MENZEL_JEMIL_CN_101404944_225000_CN_178494278_225000/RConn3 -- T_178494278__POSTE_MENZEL_JEMIL/LConn3 -- bus38/LConn1
  T_93263381__POSTE_RADES/LConn1 -- LIGNE_225_Kv_RADES_NAASAN_CN_93263381_225000_CN_125504235_225000/RConn1
  T_93263381__POSTE_RADES/LConn2 -- LIGNE_225_Kv_RADES_NAASAN_CN_93263381_225000_CN_125504235_225000/RConn2
  LIGNE_225_Kv_RADES_NAASAN_CN_93263381_225000_CN_125504235_225000/RConn3 -- T_93263381__POSTE_RADES/LConn3 -- bus39/LConn1
  T_178326515__POSTE_MOKNINE/LConn1 -- LIGNE_225_Kv_SIDI_MANSOUR_DIV_MOKNINE_CN_178328237_225000_CN_178326515_225000/RConn1
  T_178326515__POSTE_MOKNINE/LConn2 -- LIGNE_225_Kv_SIDI_MANSOUR_DIV_MOKNINE_CN_178328237_225000_CN_178326515_225000/RConn2
  LIGNE_225_Kv_SIDI_MANSOUR_DIV_MOKNINE_CN_178328237_225000_CN_178326515_225000/RConn3 -- T_178326515__POSTE_MOKNINE/LConn3 -- bus40/LConn1
  _CN_178328237_225000_CN_189193646_225000/RConn1 -- T_189193646__POSTE_BOUCHEMMA/LConn1 -- _CN_189193646_225000_CN_189193656_225000/LConn1 -- LIGNE_225_Kv_BOUCHEMMA_MEKNASSY_CN_189193646_225000_CN_201812735_225000/LConn1 -- _CN_189193646_225000_CN_180611326_225000/LConn1 -- LIGNE_225_Kv_BOUCHEMMA_TATAOUINE_CN_189193646_225000_CN_180615776_225000/LConn1
  _CN_178328237_225000_CN_189193646_225000/RConn2 -- T_189193646__POSTE_BOUCHEMMA/LConn2 -- _CN_189193646_225000_CN_189193656_225000/LConn2 -- LIGNE_225_Kv_BOUCHEMMA_MEKNASSY_CN_189193646_225000_CN_201812735_225000/LConn2 -- _CN_189193646_225000_CN_180611326_225000/LConn2 -- LIGNE_225_Kv_BOUCHEMMA_TATAOUINE_CN_189193646_225000_CN_180615776_225000/LConn2
  _CN_178328237_225000_CN_189193646_225000/RConn3 -- T_189193646__POSTE_BOUCHEMMA/LConn3 -- _CN_189193646_225000_CN_189193656_225000/LConn3 -- LIGNE_225_Kv_BOUCHEMMA_MEKNASSY_CN_189193646_225000_CN_201812735_225000/LConn3 -- _CN_189193646_225000_CN_180611326_225000/LConn3 -- LIGNE_225_Kv_BOUCHEMMA_TATAOUINE_CN_189193646_225000_CN_180615776_225000/LConn3 -- bus41/LConn1
  T_189193656__/LConn1 -- _CN_189193646_225000_CN_189193656_225000/RConn1
  T_189193656__/LConn2 -- _CN_189193646_225000_CN_189193656_225000/RConn2
  _CN_189193646_225000_CN_189193656_225000/RConn3 -- T_189193656__/LConn3 -- bus42/LConn1
  LIGNE_225_Kv_BOUCHEMMA_MEKNASSY_CN_189193646_225000_CN_201812735_225000/RConn1 -- T_201812735__POSTE_MEKNASSY/LConn1 -- LIGNE_150_Kv_MEKNASSY_HAJEB_LAYOUN_CN_224417135_225000_CN_201812735_225000/RConn1
  LIGNE_225_Kv_BOUCHEMMA_MEKNASSY_CN_189193646_225000_CN_201812735_225000/RConn2 -- T_201812735__POSTE_MEKNASSY/LConn2 -- LIGNE_150_Kv_MEKNASSY_HAJEB_LAYOUN_CN_224417135_225000_CN_201812735_225000/RConn2
  LIGNE_225_Kv_BOUCHEMMA_MEKNASSY_CN_189193646_225000_CN_201812735_225000/RConn3 -- T_201812735__POSTE_MEKNASSY/LConn3 -- LIGNE_150_Kv_MEKNASSY_HAJEB_LAYOUN_CN_224417135_225000_CN_201812735_225000/RConn3 -- bus43/LConn1
  _CN_189193646_225000_CN_180611326_225000/RConn1 -- T_180611326__POSTE_MEDENINE/LConn1 -- LIGNE_225_Kv_MEDENINE_TATAOUINE_CN_180615776_225000_CN_180611326_225000/LConn1
  _CN_189193646_225000_CN_180611326_225000/RConn2 -- T_180611326__POSTE_MEDENINE/LConn2 -- LIGNE_225_Kv_MEDENINE_TATAOUINE_CN_180615776_225000_CN_180611326_225000/LConn2
  _CN_189193646_225000_CN_180611326_225000/RConn3 -- T_180611326__POSTE_MEDENINE/LConn3 -- LIGNE_225_Kv_MEDENINE_TATAOUINE_CN_180615776_225000_CN_180611326_225000/LConn3 -- bus44/LConn1
  LIGNE_225_Kv_BOUCHEMMA_TATAOUINE_CN_189193646_225000_CN_180615776_225000/RConn1 -- T_180615776__POSTE_TATAOUINE/LConn1 -- LIGNE_225_Kv_MEDENINE_TATAOUINE_CN_180615776_225000_CN_180611326_225000/RConn1
  LIGNE_225_Kv_BOUCHEMMA_TATAOUINE_CN_189193646_225000_CN_180615776_225000/RConn2 -- T_180615776__POSTE_TATAOUINE/LConn2 -- LIGNE_225_Kv_MEDENINE_TATAOUINE_CN_180615776_225000_CN_180611326_225000/RConn2
  LIGNE_225_Kv_BOUCHEMMA_TATAOUINE_CN_189193646_225000_CN_180615776_225000/RConn3 -- T_180615776__POSTE_TATAOUINE/LConn3 -- LIGNE_225_Kv_MEDENINE_TATAOUINE_CN_180615776_225000_CN_180611326_225000/RConn3 -- bus45/LConn1
  T_242398869__POSTE_KAIROUAN/LConn1 -- LIGNE_225_Kv_KAIROUAN_CIMENTERIE_CN_242398869_225000_CN_226848748_225000/LConn1
  T_242398869__POSTE_KAIROUAN/LConn2 -- LIGNE_225_Kv_KAIROUAN_CIMENTERIE_CN_242398869_225000_CN_226848748_225000/LConn2
  LIGNE_225_Kv_KAIROUAN_CIMENTERIE_CN_242398869_225000_CN_226848748_225000/LConn3 -- T_242398869__POSTE_KAIROUAN/LConn3 -- bus46/LConn1
  T_226848748__/LConn1 -- LIGNE_225_Kv_KAIROUAN_CIMENTERIE_CN_242398869_225000_CN_226848748_225000/RConn1
  T_226848748__/LConn2 -- LIGNE_225_Kv_KAIROUAN_CIMENTERIE_CN_242398869_225000_CN_226848748_225000/RConn2
  LIGNE_225_Kv_KAIROUAN_CIMENTERIE_CN_242398869_225000_CN_226848748_225000/RConn3 -- T_226848748__/LConn3 -- bus47/LConn1
  T_106469430__POSTE_BOUFICHA/LConn1 -- LIGNE_225_Kv__BOUFICHA_ZAGHOUAN_CN_106469430_225000_CN_173531194_225000/RConn1
  T_106469430__POSTE_BOUFICHA/LConn2 -- LIGNE_225_Kv__BOUFICHA_ZAGHOUAN_CN_106469430_225000_CN_173531194_225000/RConn2
  LIGNE_225_Kv__BOUFICHA_ZAGHOUAN_CN_106469430_225000_CN_173531194_225000/RConn3 -- T_106469430__POSTE_BOUFICHA/LConn3 -- bus48/LConn1
  T_130775787__POSTE_MSAKEN/RConn1 -- L_130775787/LConn1
  T_130775787__POSTE_MSAKEN/RConn2 -- L_130775787/LConn2
  L_130775787/LConn3 -- T_130775787__POSTE_MSAKEN/RConn3 -- bus49/LConn1
  T_111375430__/RConn1 -- L_111375430/LConn1
  T_111375430__/RConn2 -- L_111375430/LConn2
  L_111375430/LConn3 -- T_111375430__/RConn3 -- bus50/LConn1
  T_178543491__POSTE_GREMDA/RConn1 -- L_178543491/LConn1
  T_178543491__POSTE_GREMDA/RConn2 -- L_178543491/LConn2
  L_178543491/LConn3 -- T_178543491__POSTE_GREMDA/RConn3 -- bus51/LConn1
  T_178549814__POSTE_ELJEM/RConn1 -- L_178549814/LConn1
  T_178549814__POSTE_ELJEM/RConn2 -- L_178549814/LConn2
  L_178549814/LConn3 -- T_178549814__POSTE_ELJEM/RConn3 -- bus52/LConn1
  T_178547287__POSTE_THYNA/RConn1 -- L_178547287/LConn1
  T_178547287__POSTE_THYNA/RConn2 -- L_178547287/LConn2
  L_178547287/LConn3 -- T_178547287__POSTE_THYNA/RConn3 -- bus53/LConn1
  T_322419513__POSTE_DE_LA_CIMENTERIE_DE_GABES/RConn1 -- L_322419513/LConn1
  T_322419513__POSTE_DE_LA_CIMENTERIE_DE_GABES/RConn2 -- L_322419513/LConn2
  L_322419513/LConn3 -- T_322419513__POSTE_DE_LA_CIMENTERIE_DE_GABES/RConn3 -- bus54/LConn1
  T_202286224__POSTE_SKHIRA/RConn1 -- L_202286224/LConn1
  T_202286224__POSTE_SKHIRA/RConn2 -- L_202286224/LConn2
  L_202286224/LConn3 -- T_202286224__POSTE_SKHIRA/RConn3 -- bus55/LConn1
  T_242390602__POSTE_DE_GHANNOUCH/RConn1 -- L_242390602/LConn1
  T_242390602__POSTE_DE_GHANNOUCH/RConn2 -- L_242390602/LConn2
  L_242390602/LConn3 -- T_242390602__POSTE_DE_GHANNOUCH/RConn3 -- bus56/LConn1
  T_252371715__POSTE_FERIANA/RConn1 -- L_252371715/LConn1
  T_252371715__POSTE_FERIANA/RConn2 -- L_252371715/LConn2
  L_252371715/LConn3 -- T_252371715__POSTE_FERIANA/RConn3 -- bus57/LConn1
  T_206449367_150000_POSTE_DE_MDHILLA/RConn1 -- L_206449367/LConn1
  T_206449367_150000_POSTE_DE_MDHILLA/RConn2 -- L_206449367/LConn2
  L_206449367/LConn3 -- T_206449367_150000_POSTE_DE_MDHILLA/RConn3 -- bus58/LConn1
  T_206389818__POSTE_METLAOUI/RConn1 -- L_206389818/LConn1
  T_206389818__POSTE_METLAOUI/RConn2 -- L_206389818/LConn2
  L_206389818/LConn3 -- T_206389818__POSTE_METLAOUI/RConn3 -- bus59/LConn1
  T_207339172__POSTE_TOZEUR/RConn1 -- L_207339172/LConn1
  T_207339172__POSTE_TOZEUR/RConn2 -- L_207339172/LConn2
  L_207339172/LConn3 -- T_207339172__POSTE_TOZEUR/RConn3 -- bus60/LConn1
  T_174150822__POSTE_LESSOUDA/RConn1 -- L_174150822/LConn1
  T_174150822__POSTE_LESSOUDA/RConn2 -- L_174150822/LConn2
  L_174150822/LConn3 -- T_174150822__POSTE_LESSOUDA/RConn3 -- bus61/LConn1
  T_131220525__Poste__Enfidha_Sud/RConn1 -- L_131220525/LConn1
  T_131220525__Poste__Enfidha_Sud/RConn2 -- L_131220525/LConn2
  L_131220525/LConn3 -- T_131220525__Poste__Enfidha_Sud/RConn3 -- bus62/LConn1
  T_242392536__POSTE_GABES_SUD/RConn1 -- L_242392536/LConn1
  T_242392536__POSTE_GABES_SUD/RConn2 -- L_242392536/LConn2
  L_242392536/LConn3 -- T_242392536__POSTE_GABES_SUD/RConn3 -- bus63/LConn1
  T_253586233__POSTE_DE_KEBILI/RConn1 -- L_253586233/LConn1
  T_253586233__POSTE_DE_KEBILI/RConn2 -- L_253586233/LConn2
  L_253586233/LConn3 -- T_253586233__POSTE_DE_KEBILI/RConn3 -- bus64/LConn1
